simulink model "Supported_and_unsupported_combinations"  (Simulink 7.8)
settings: Solver=ode15s  StartTime=0.0  StopTime=inf  MaxStep=0.2  RelTol=1e-3
undefined symbols (not defined in the file): Engine, Engine1, Engine2, Engine3, Engine4, Engine5, Engine6, Engine7, Engine8, Engine9
libraries: sFunctionBlocks x32
(part 1 of 4)
settings Model: Creator=e675225  LastModifiedBy=e675225
settings DebuggingCC: UnconnectedLineMsg=none

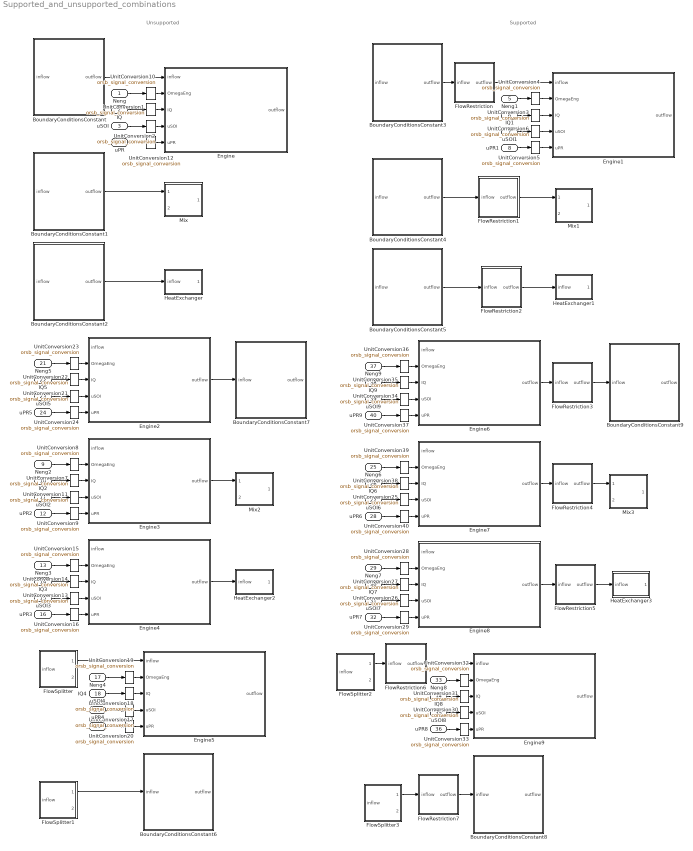
== system Supported_and_unsupported_combinations ==
  note: Unsupported
  note: Supported
  Neng : Inport
  IQ : Inport  Port=2
  uSOI : Inport  Tag=actuator  Port=3
  uPR : Inport  Port=4
  Neng1 : Inport  Port=5
  IQ1 : Inport  Port=6
  uSOI1 : Inport  Tag=actuator  Port=7
  uPR1 : Inport  Port=8
  Neng2 : Inport  Port=9
  IQ2 : Inport  Port=10
  uSOI2 : Inport  Tag=actuator  Port=11
  uPR2 : Inport  Port=12
  Neng3 : Inport  Port=13
  IQ3 : Inport  Port=14
  uSOI3 : Inport  Tag=actuator  Port=15
  uPR3 : Inport  Port=16
  Neng4 : Inport  Port=17
  IQ4 : Inport  Port=18
  uSOI4 : Inport  Tag=actuator  Port=19
  uPR4 : Inport  Port=20
  Neng5 : Inport  Port=21
  IQ5 : Inport  Port=22
  uSOI5 : Inport  Tag=actuator  Port=23
  uPR5 : Inport  Port=24
  Neng6 : Inport  Port=25
  IQ6 : Inport  Port=26
  uSOI6 : Inport  Tag=actuator  Port=27
  uPR6 : Inport  Port=28
  Neng7 : Inport  Port=29
  IQ7 : Inport  Port=30
  uSOI7 : Inport  Tag=actuator  Port=31
  uPR7 : Inport  Port=32
  Neng8 : Inport  Port=33
  IQ8 : Inport  Port=34
  uSOI8 : Inport  Tag=actuator  Port=35
  uPR8 : Inport  Port=36
  Neng9 : Inport  Port=37
  IQ9 : Inport  Port=38
  uSOI9 : Inport  Tag=actuator  Port=39
  uPR9 : Inport  Port=40
  BoundaryConditionsConstant : Subsystem  mask(amb_conditions){XO2bc=0.231362, Tbc=293, Pbc=1e5}
      mask prompts: XO2bc "<b>XO2bc:</b> boundary condition oxygen mass fraction [-]"; Tbc "<b>Tbc:</b> boundary condition temperature [K]"; Pbc "<b>Pbc:</b> boundary condition pressure [Pa]"
      mask Display:
      | plot([0], [-0.5])
      | plot([1], [0.5])
      | plot((0.1:0.01:0.87), sqrt(0.8*((0.1:0.01:0.87)-0.1)-((0.1:0.01:0.87)-0.1).^2))
      | plot((0.1:0.01:0.87), -sqrt(0.8*((0.1:0.01:0.87)-0.1)-((0.1:0.01:0.87)-0.1).^2))
      | plot([0.87 0.95], sqrt(0.8*((0.87)-0.1)-((0.87)-0.1).^2)*[1 1])
      | plot([0.87 0.95], -sqrt(0.8*((0.87)-0.1)-((0.87)-0.1).^2)*[1 1])
  BoundaryConditionsConstant1 : Subsystem  mask(amb_conditions){XO2bc=0.231362, Tbc=293, Pbc=1e5}
      mask prompts: XO2bc "<b>XO2bc:</b> boundary condition oxygen mass fraction [-]"; Tbc "<b>Tbc:</b> boundary condition temperature [K]"; Pbc "<b>Pbc:</b> boundary condition pressure [Pa]"
      mask Display:
      | plot([0], [-0.5])
      | plot([1], [0.5])
      | plot((0.1:0.01:0.87), sqrt(0.8*((0.1:0.01:0.87)-0.1)-((0.1:0.01:0.87)-0.1).^2))
      | plot((0.1:0.01:0.87), -sqrt(0.8*((0.1:0.01:0.87)-0.1)-((0.1:0.01:0.87)-0.1).^2))
      | plot([0.87 0.95], sqrt(0.8*((0.87)-0.1)-((0.87)-0.1).^2)*[1 1])
      | plot([0.87 0.95], -sqrt(0.8*((0.87)-0.1)-((0.87)-0.1).^2)*[1 1])
  BoundaryConditionsConstant2 : Subsystem  mask(amb_conditions){XO2bc=0.231362, Tbc=293, Pbc=1e5}
      mask prompts: XO2bc "<b>XO2bc:</b> boundary condition oxygen mass fraction [-]"; Tbc "<b>Tbc:</b> boundary condition temperature [K]"; Pbc "<b>Pbc:</b> boundary condition pressure [Pa]"
      mask Display:
      | plot([0], [-0.5])
      | plot([1], [0.5])
      | plot((0.1:0.01:0.87), sqrt(0.8*((0.1:0.01:0.87)-0.1)-((0.1:0.01:0.87)-0.1).^2))
      | plot((0.1:0.01:0.87), -sqrt(0.8*((0.1:0.01:0.87)-0.1)-((0.1:0.01:0.87)-0.1).^2))
      | plot([0.87 0.95], sqrt(0.8*((0.87)-0.1)-((0.87)-0.1).^2)*[1 1])
      | plot([0.87 0.95], -sqrt(0.8*((0.87)-0.1)-((0.87)-0.1).^2)*[1 1])
  BoundaryConditionsConstant3 : Subsystem  mask(amb_conditions){XO2bc=0.231362, Tbc=293, Pbc=1e5}
      mask prompts: XO2bc "<b>XO2bc:</b> boundary condition oxygen mass fraction [-]"; Tbc "<b>Tbc:</b> boundary condition temperature [K]"; Pbc "<b>Pbc:</b> boundary condition pressure [Pa]"
      mask Display:
      | plot([0], [-0.5])
      | plot([1], [0.5])
      | plot((0.1:0.01:0.87), sqrt(0.8*((0.1:0.01:0.87)-0.1)-((0.1:0.01:0.87)-0.1).^2))
      | plot((0.1:0.01:0.87), -sqrt(0.8*((0.1:0.01:0.87)-0.1)-((0.1:0.01:0.87)-0.1).^2))
      | plot([0.87 0.95], sqrt(0.8*((0.87)-0.1)-((0.87)-0.1).^2)*[1 1])
      | plot([0.87 0.95], -sqrt(0.8*((0.87)-0.1)-((0.87)-0.1).^2)*[1 1])
  BoundaryConditionsConstant4 : Subsystem  mask(amb_conditions){XO2bc=0.231362, Tbc=293, Pbc=1e5}
      mask prompts: XO2bc "<b>XO2bc:</b> boundary condition oxygen mass fraction [-]"; Tbc "<b>Tbc:</b> boundary condition temperature [K]"; Pbc "<b>Pbc:</b> boundary condition pressure [Pa]"
      mask Display:
      | plot([0], [-0.5])
      | plot([1], [0.5])
      | plot((0.1:0.01:0.87), sqrt(0.8*((0.1:0.01:0.87)-0.1)-((0.1:0.01:0.87)-0.1).^2))
      | plot((0.1:0.01:0.87), -sqrt(0.8*((0.1:0.01:0.87)-0.1)-((0.1:0.01:0.87)-0.1).^2))
      | plot([0.87 0.95], sqrt(0.8*((0.87)-0.1)-((0.87)-0.1).^2)*[1 1])
      | plot([0.87 0.95], -sqrt(0.8*((0.87)-0.1)-((0.87)-0.1).^2)*[1 1])
  BoundaryConditionsConstant5 : Subsystem  mask(amb_conditions){XO2bc=0.231362, Tbc=293, Pbc=1e5}
      mask prompts: XO2bc "<b>XO2bc:</b> boundary condition oxygen mass fraction [-]"; Tbc "<b>Tbc:</b> boundary condition temperature [K]"; Pbc "<b>Pbc:</b> boundary condition pressure [Pa]"
      mask Display:
      | plot([0], [-0.5])
      | plot([1], [0.5])
      | plot((0.1:0.01:0.87), sqrt(0.8*((0.1:0.01:0.87)-0.1)-((0.1:0.01:0.87)-0.1).^2))
      | plot((0.1:0.01:0.87), -sqrt(0.8*((0.1:0.01:0.87)-0.1)-((0.1:0.01:0.87)-0.1).^2))
      | plot([0.87 0.95], sqrt(0.8*((0.87)-0.1)-((0.87)-0.1).^2)*[1 1])
      | plot([0.87 0.95], -sqrt(0.8*((0.87)-0.1)-((0.87)-0.1).^2)*[1 1])
  BoundaryConditionsConstant6 : Subsystem  mask(amb_conditions){XO2bc=0.231362, Tbc=293, Pbc=1e5}
      mask prompts: XO2bc "<b>XO2bc:</b> boundary condition oxygen mass fraction [-]"; Tbc "<b>Tbc:</b> boundary condition temperature [K]"; Pbc "<b>Pbc:</b> boundary condition pressure [Pa]"
      mask Display:
      | plot([0], [-0.5])
      | plot([1], [0.5])
      | plot((0.1:0.01:0.87), sqrt(0.8*((0.1:0.01:0.87)-0.1)-((0.1:0.01:0.87)-0.1).^2))
      | plot((0.1:0.01:0.87), -sqrt(0.8*((0.1:0.01:0.87)-0.1)-((0.1:0.01:0.87)-0.1).^2))
      | plot([0.87 0.95], sqrt(0.8*((0.87)-0.1)-((0.87)-0.1).^2)*[1 1])
      | plot([0.87 0.95], -sqrt(0.8*((0.87)-0.1)-((0.87)-0.1).^2)*[1 1])
  BoundaryConditionsConstant7 : Subsystem  mask(amb_conditions){XO2bc=0.231362, Tbc=293, Pbc=1e5}
      mask prompts: XO2bc "<b>XO2bc:</b> boundary condition oxygen mass fraction [-]"; Tbc "<b>Tbc:</b> boundary condition temperature [K]"; Pbc "<b>Pbc:</b> boundary condition pressure [Pa]"
      mask Display:
      | plot([0], [-0.5])
      | plot([1], [0.5])
      | plot((0.1:0.01:0.87), sqrt(0.8*((0.1:0.01:0.87)-0.1)-((0.1:0.01:0.87)-0.1).^2))
      | plot((0.1:0.01:0.87), -sqrt(0.8*((0.1:0.01:0.87)-0.1)-((0.1:0.01:0.87)-0.1).^2))
      | plot([0.87 0.95], sqrt(0.8*((0.87)-0.1)-((0.87)-0.1).^2)*[1 1])
      | plot([0.87 0.95], -sqrt(0.8*((0.87)-0.1)-((0.87)-0.1).^2)*[1 1])
  BoundaryConditionsConstant8 : Subsystem  mask(amb_conditions){XO2bc=0.231362, Tbc=293, Pbc=1e5}
      mask prompts: XO2bc "<b>XO2bc:</b> boundary condition oxygen mass fraction [-]"; Tbc "<b>Tbc:</b> boundary condition temperature [K]"; Pbc "<b>Pbc:</b> boundary condition pressure [Pa]"
      mask Display:
      | plot([0], [-0.5])
      | plot([1], [0.5])
      | plot((0.1:0.01:0.87), sqrt(0.8*((0.1:0.01:0.87)-0.1)-((0.1:0.01:0.87)-0.1).^2))
      | plot((0.1:0.01:0.87), -sqrt(0.8*((0.1:0.01:0.87)-0.1)-((0.1:0.01:0.87)-0.1).^2))
      | plot([0.87 0.95], sqrt(0.8*((0.87)-0.1)-((0.87)-0.1).^2)*[1 1])
      | plot([0.87 0.95], -sqrt(0.8*((0.87)-0.1)-((0.87)-0.1).^2)*[1 1])
  BoundaryConditionsConstant9 : Subsystem  mask(amb_conditions){XO2bc=0.231362, Tbc=293, Pbc=1e5}
      mask prompts: XO2bc "<b>XO2bc:</b> boundary condition oxygen mass fraction [-]"; Tbc "<b>Tbc:</b> boundary condition temperature [K]"; Pbc "<b>Pbc:</b> boundary condition pressure [Pa]"
      mask Display:
      | plot([0], [-0.5])
      | plot([1], [0.5])
      | plot((0.1:0.01:0.87), sqrt(0.8*((0.1:0.01:0.87)-0.1)-((0.1:0.01:0.87)-0.1).^2))
      | plot((0.1:0.01:0.87), -sqrt(0.8*((0.1:0.01:0.87)-0.1)-((0.1:0.01:0.87)-0.1).^2))
      | plot([0.87 0.95], sqrt(0.8*((0.87)-0.1)-((0.87)-0.1).^2)*[1 1])
      | plot([0.87 0.95], -sqrt(0.8*((0.87)-0.1)-((0.87)-0.1).^2)*[1 1])
  Engine : Subsystem  mask(engine_subsys){setOutportFuel_Massflow=off, nameOutportFuel_Massflow=Fuel_Massflow_Engine, setOutportEngine_Speed=off, nameOutportEngine_Speed=Omega_Engine, setOutportCylinder_Pressure=off, nameOutportCylinder_Pressure=Pressure_in_cylinder_Engine, blockName=Engine}
      mask prompts: setOutportFuel_Massflow "readout fuel mass flow [kg/s]"; nameOutportFuel_Massflow "variable name to readout fuel mass flow"; setOutportEngine_Speed "readout engine speed [rad/s]"; nameOutportEngine_Speed "variable name to readout engine speed"; setOutportCylinder_Pressure "readout cylinder pressure [Pa]"; nameOutportCylinder_Pressure "variable name to readout cylinder pressure"; blockName "name of readout block (internal use only)"
      mask init:
      | %Speed icon
      | if setOutportEngine_Speed
      |     r = 0.08;
      |     xCenter = 0.5;
      |     yCenter = 0.2;
      |     xSpeed1 = [0.53 0.5 0.53];                          ySpeed1 = yCenter - 1*(r + [0.04 0 -0.04]);
      |     xSpeed2 = ((xCenter-r) : 0.001 :(xCenter + r)); ySpeed2 = yCenter + 1*sqrt(abs(r^2-(xSpeed2-xCenter).^2));
      |     xSpeed3 = xSpeed2;                              ySpeed3 = yCenter - 1*sqrt(abs(r^2-(xSpeed3-xCenter).^2));
      | else
      |     xSpeed1 = 0;   ySpeed1 = 0;
      |     xSpeed2 = 0;   ySpeed2 = 0;
      |     xSpeed3 = 0;   ySpeed3 = 0;
      | end
      | 
      | 
      | %Massflow icon
      | if setOutportFuel_Massflow
      |     xFlow1 = [0.45 0.45]; yFlow1 = [0.95 0.85];
      |     xFlow2 = [0.55 0.55];	yFlow2 = yFlow1;
      |     xFlow3 = [0.5 0.5];	yFlow3 = [0.97 0.83];
      |     xFlow4 = [0.49 0.5 0.51];    yFlow4 = [0.87 0.83 0.87];
      | else
      |     xFlow1 = 0;    yFlow1 = 0;
      |     xFlow2 = 0;    yFlow2 = 0;
      |     xFlow3 = 0;    yFlow3 = 0;
      |     xFlow4 = 0;    yFlow4 = 0;
      | end
      | 
      | 
      | %Pressure icon
      | if setOutportCylinder_Pressure
      |     r = 0.06;
      |     xCenter = 0.5;
      |     yCenter = 1.1;
      |     xPress1 = [xCenter-r xCenter+r];                yPress1 = [yCenter-r yCenter+r];
      |     xPress2 = [xCenter+r-r/4 xCenter+r xCenter+r];  yPress2 = [yCenter+r yCenter+r yCenter+r-r/4];
      |     xPress3 = ((xCenter-r) : 0.001 :(xCenter + r)); yPress3 = yCenter + sqrt(abs(r^2-(xPress3-xCenter).^2));
      |     xPress4 = xPress3;                              yPress4 = yCenter - sqrt(abs(r^2-(xPress4-xCenter).^2));
      | else
      |     xPress1 = 0;   yPress1 = 0;
      |     xPress2 = 0;   yPress2 = 0;
      |     xPress3 = 0;   yPress3 = 0;
      |     xPress4 = 0;   yPress4 = 0;
      | end
      settings: CopyFcn=|
      | set_param(gcb, 'blockName', get_param(gcb, 'Name'))
      | set_param(gcb, 'setOutportFuel_Massflow', 'off')
      | set_param(gcb, 'nameOutportFuel_Massflow', ['Fuel_Massflow_' get_param(gcb, 'blockName')])
      | set_param(gcb, 'setOutportEngine_Speed', 'off')
      | set_param(gcb, 'nameOutportEngine_Speed', ['Omega_' get_param(gcb, 'blockName')])
      | set_param(gcb, 'setOutportCylinder_Pressure', 'off')
      | set_param(gcb, 'nameOutportCylinder_Pressure', ['Pressure_in_cylinder_' get_param(gcb, 'blockName')])
      settings: NameChangeFcn=|
      | %if variable name is default change this name on name change of block
      | 
      | 
      | if strcmp(get_param(gcb, 'nameOutportFuel_Massflow'), [ 'Fuel_Massflow_' get_param(gcb, 'blockName') ])
      | set_param(gcb, 'nameOutportFuel_Massflow', ['Fuel_Massflow_' get_param(gcb, 'Name')])
      | end
      | 
      | 
      | 
      | 
      | if strcmp(get_param(gcb, 'nameOutportEngine_Speed'), [ 'Omega_' get_param(gcb, 'blockName') ])
      | set_param(gcb, 'nameOutportEngine_Speed', ['Omega_' get_param(gcb, 'Name')])
      | end
      | 
      | 
      | set_param(gcb, 'blockName', get_param(gcb, 'Name'))
      mask CallbackString:
      | en = get_param(gcb,'MaskEnables');
      | 
      | switch get_param(gcb,'setOutportFuel_Massflow')
      | 
      |     case 'on'
      |         en{2} = 'on';
      |     case 'off'
      |         en{2} = 'off';
      | end
      | 
      | set_param(gcb,'MaskEnables',en)|%% Check for empty strings
      | if isempty(strtrim(get_param(gcb, 'nameOutportFuel_Massflow')))
      |     set_param(gcb, 'nameOutportFuel_Massflow', ['Fuel_Massflow_' get_param(gcb, 'Name')])
      |     error('Empty string for readout variable not allowed')
      | end
      | 
      | 
      | %% Check for repeated outport names
      | checkOutportName('nameOutportFuel_Massflow', 'Fuel_Massflow')|en = get_param(gcb,'MaskEnables');
      | 
      | switch get_param(gcb,'setOutportEngine_Speed')
      | 
      |     case 'on'
      |         en{4} = 'on';
      |     case 'off'
      |         en{4} = 'off';
      | end
      | 
      | set_param(gcb,'MaskEnables',en)|%% Check for empty strings
      | if isempty(strtrim(get_param(gcb, 'nameOutportEngine_Speed')))
      |     set_param(gcb, 'nameOutportEngine_Speed', ['Engine_Speed_' get_param(gcb, 'Name')])
      |     error('Empty string for readout variable not allowed')
      | end
      | 
      | 
      | %% Check for repeated outport names
      | checkOutportName('nameOutportEngine_Speed', 'Engine_Speed')|en = get_param(gcb,'MaskEnables');
      | 
      | switch get_param(gcb,'setOutportCylinder_Pressure')
      | 
      |     case 'on'
      |         en{6} = 'on';
      |     case 'off'
      |         en{6} = 'off';
      | end
      | 
      | set_param(gcb,'MaskEnables',en)|%% Check for empty strings
      | if isempty(strtrim(get_param(gcb, 'nameOutportFuel_Massflow')))
      |     set_param(gcb, 'nameOutportFuel_Massflow', ['Fuel_Massflow_' get_param(gcb, 'Name')])
      |     error('Empty string for readout variable not allowed')
      | end
      | 
      | 
      | %% Check for repeated outport names
      | checkOutportName('nameOutportFuel_Massflow', 'Fuel_Massflow')|
      mask Display:
      | plot([-0.1], [-0.1])
      | plot([1.1], [1.1])
      | plot([0.18,0.18],[0,1])
      | plot([0.21,0.21],[0,1])
      | plot([0.82,0.82],[0,1])
      | plot([0.79,0.79],[0,1])
      | plot([0.22,0.22,0.3, 0.7, 0.78, 0.78, 0.22],[0.8, 0.4, 0.35, 0.35, 0.4,0.8,0.8])
      | plot([0.21,0.79],[0.7,0.7])
      | plot([0.21,0.79],[0.66,0.66])
      | plot([0.21,0.79],[0.7,0.7])
      | plot([0.47,0.6],[0.35,0])
      | plot([0.53,0.66],[0.35,0])
      | 
      | color('green');
      | plot(xSpeed1, ySpeed1)
      | plot(xSpeed2, ySpeed2)
      | plot(xSpeed3, ySpeed3)
      | 
      | color('magenta');
      | plot(xFlow1, yFlow1)
      | plot(xFlow2, yFlow2)
      | plot(xFlow3, yFlow3)
      | plot(xFlow4, yFlow4)
      | 
      | color('blue');
      | plot(xPress1, yPress1)
      | plot(xPress2, yPress2)
      | plot(xPress3, yPress3)
      | plot(xPress4, yPress4)
  Engine1 : Subsystem  mask(engine_subsys){setOutportFuel_Massflow=off, nameOutportFuel_Massflow=Fuel_Massflow_Engine1, setOutportEngine_Speed=off, nameOutportEngine_Speed=Omega_Engine1, setOutportCylinder_Pressure=off, nameOutportCylinder_Pressure=Pressure_in_cylinder_Engine1, blockName=Engine1}
      mask prompts: setOutportFuel_Massflow "readout fuel mass flow [kg/s]"; nameOutportFuel_Massflow "variable name to readout fuel mass flow"; setOutportEngine_Speed "readout engine speed [rad/s]"; nameOutportEngine_Speed "variable name to readout engine speed"; setOutportCylinder_Pressure "readout cylinder pressure [Pa]"; nameOutportCylinder_Pressure "variable name to readout cylinder pressure"; blockName "name of readout block (internal use only)"
      mask init: same as Supported_and_unsupported_combinations/Engine
      settings: CopyFcn=|
      | set_param(gcb, 'blockName', get_param(gcb, 'Name'))
      | set_param(gcb, 'setOutportFuel_Massflow', 'off')
      | set_param(gcb, 'nameOutportFuel_Massflow', ['Fuel_Massflow_' get_param(gcb, 'blockName')])
      | set_param(gcb, 'setOutportEngine_Speed', 'off')
      | set_param(gcb, 'nameOutportEngine_Speed', ['Omega_' get_param(gcb, 'blockName')])
      | set_param(gcb, 'setOutportCylinder_Pressure', 'off')
      | set_param(gcb, 'nameOutportCylinder_Pressure', ['Pressure_in_cylinder_' get_param(gcb, 'blockName')])
      settings: NameChangeFcn=|
      | %if variable name is default change this name on name change of block
      | 
      | 
      | if strcmp(get_param(gcb, 'nameOutportFuel_Massflow'), [ 'Fuel_Massflow_' get_param(gcb, 'blockName') ])
      | set_param(gcb, 'nameOutportFuel_Massflow', ['Fuel_Massflow_' get_param(gcb, 'Name')])
      | end
      | 
      | 
      | 
      | 
      | if strcmp(get_param(gcb, 'nameOutportEngine_Speed'), [ 'Omega_' get_param(gcb, 'blockName') ])
      | set_param(gcb, 'nameOutportEngine_Speed', ['Omega_' get_param(gcb, 'Name')])
      | end
      | 
      | 
      | set_param(gcb, 'blockName', get_param(gcb, 'Name'))
      mask CallbackString:
      | en = get_param(gcb,'MaskEnables');
      | 
      | switch get_param(gcb,'setOutportFuel_Massflow')
      | 
      |     case 'on'
      |         en{2} = 'on';
      |     case 'off'
      |         en{2} = 'off';
      | end
      | 
      | set_param(gcb,'MaskEnables',en)|%% Check for empty strings
      | if isempty(strtrim(get_param(gcb, 'nameOutportFuel_Massflow')))
      |     set_param(gcb, 'nameOutportFuel_Massflow', ['Fuel_Massflow_' get_param(gcb, 'Name')])
      |     error('Empty string for readout variable not allowed')
      | end
      | 
      | 
      | %% Check for repeated outport names
      | checkOutportName('nameOutportFuel_Massflow', 'Fuel_Massflow')|en = get_param(gcb,'MaskEnables');
      | 
      | switch get_param(gcb,'setOutportEngine_Speed')
      | 
      |     case 'on'
      |         en{4} = 'on';
      |     case 'off'
      |         en{4} = 'off';
      | end
      | 
      | set_param(gcb,'MaskEnables',en)|%% Check for empty strings
      | if isempty(strtrim(get_param(gcb, 'nameOutportEngine_Speed')))
      |     set_param(gcb, 'nameOutportEngine_Speed', ['Engine_Speed_' get_param(gcb, 'Name')])
      |     error('Empty string for readout variable not allowed')
      | end
      | 
      | 
      | %% Check for repeated outport names
      | checkOutportName('nameOutportEngine_Speed', 'Engine_Speed')|en = get_param(gcb,'MaskEnables');
      | 
      | switch get_param(gcb,'setOutportCylinder_Pressure')
      | 
      |     case 'on'
      |         en{6} = 'on';
      |     case 'off'
      |         en{6} = 'off';
      | end
      | 
      | set_param(gcb,'MaskEnables',en)|%% Check for empty strings
      | if isempty(strtrim(get_param(gcb, 'nameOutportFuel_Massflow')))
      |     set_param(gcb, 'nameOutportFuel_Massflow', ['Fuel_Massflow_' get_param(gcb, 'Name')])
      |     error('Empty string for readout variable not allowed')
      | end
      | 
      | 
      | %% Check for repeated outport names
      | checkOutportName('nameOutportFuel_Massflow', 'Fuel_Massflow')|
      mask Display:
      | plot([-0.1], [-0.1])
      | plot([1.1], [1.1])
      | plot([0.18,0.18],[0,1])
      | plot([0.21,0.21],[0,1])
      | plot([0.82,0.82],[0,1])
      | plot([0.79,0.79],[0,1])
      | plot([0.22,0.22,0.3, 0.7, 0.78, 0.78, 0.22],[0.8, 0.4, 0.35, 0.35, 0.4,0.8,0.8])
      | plot([0.21,0.79],[0.7,0.7])
      | plot([0.21,0.79],[0.66,0.66])
      | plot([0.21,0.79],[0.7,0.7])
      | plot([0.47,0.6],[0.35,0])
      | plot([0.53,0.66],[0.35,0])
      | 
      | color('green');
      | plot(xSpeed1, ySpeed1)
      | plot(xSpeed2, ySpeed2)
      | plot(xSpeed3, ySpeed3)
      | 
      | color('magenta');
      | plot(xFlow1, yFlow1)
      | plot(xFlow2, yFlow2)
      | plot(xFlow3, yFlow3)
      | plot(xFlow4, yFlow4)
      | 
      | color('blue');
      | plot(xPress1, yPress1)
      | plot(xPress2, yPress2)
      | plot(xPress3, yPress3)
      | plot(xPress4, yPress4)
  Engine2 : Subsystem  mask(engine_subsys){setOutportFuel_Massflow=off, nameOutportFuel_Massflow=Fuel_Massflow_Engine2, setOutportEngine_Speed=off, nameOutportEngine_Speed=Omega_Engine2, setOutportCylinder_Pressure=off, nameOutportCylinder_Pressure=Pressure_in_cylinder_Engine5, blockName=Engine2}
      mask prompts: setOutportFuel_Massflow "readout fuel mass flow [kg/s]"; nameOutportFuel_Massflow "variable name to readout fuel mass flow"; setOutportEngine_Speed "readout engine speed [rad/s]"; nameOutportEngine_Speed "variable name to readout engine speed"; setOutportCylinder_Pressure "readout cylinder pressure [Pa]"; nameOutportCylinder_Pressure "variable name to readout cylinder pressure"; blockName "name of readout block (internal use only)"
      mask init: same as Supported_and_unsupported_combinations/Engine
      settings: CopyFcn=|
      | set_param(gcb, 'blockName', get_param(gcb, 'Name'))
      | set_param(gcb, 'setOutportFuel_Massflow', 'off')
      | set_param(gcb, 'nameOutportFuel_Massflow', ['Fuel_Massflow_' get_param(gcb, 'blockName')])
      | set_param(gcb, 'setOutportEngine_Speed', 'off')
      | set_param(gcb, 'nameOutportEngine_Speed', ['Omega_' get_param(gcb, 'blockName')])
      | set_param(gcb, 'setOutportCylinder_Pressure', 'off')
      | set_param(gcb, 'nameOutportCylinder_Pressure', ['Pressure_in_cylinder_' get_param(gcb, 'blockName')])
      settings: NameChangeFcn=|
      | %if variable name is default change this name on name change of block
      | 
      | 
      | if strcmp(get_param(gcb, 'nameOutportFuel_Massflow'), [ 'Fuel_Massflow_' get_param(gcb, 'blockName') ])
      | set_param(gcb, 'nameOutportFuel_Massflow', ['Fuel_Massflow_' get_param(gcb, 'Name')])
      | end
      | 
      | 
      | 
      | 
      | if strcmp(get_param(gcb, 'nameOutportEngine_Speed'), [ 'Omega_' get_param(gcb, 'blockName') ])
      | set_param(gcb, 'nameOutportEngine_Speed', ['Omega_' get_param(gcb, 'Name')])
      | end
      | 
      | 
      | set_param(gcb, 'blockName', get_param(gcb, 'Name'))
      mask CallbackString:
      | en = get_param(gcb,'MaskEnables');
      | 
      | switch get_param(gcb,'setOutportFuel_Massflow')
      | 
      |     case 'on'
      |         en{2} = 'on';
      |     case 'off'
      |         en{2} = 'off';
      | end
      | 
      | set_param(gcb,'MaskEnables',en)|%% Check for empty strings
      | if isempty(strtrim(get_param(gcb, 'nameOutportFuel_Massflow')))
      |     set_param(gcb, 'nameOutportFuel_Massflow', ['Fuel_Massflow_' get_param(gcb, 'Name')])
      |     error('Empty string for readout variable not allowed')
      | end
      | 
      | 
      | %% Check for repeated outport names
      | checkOutportName('nameOutportFuel_Massflow', 'Fuel_Massflow')|en = get_param(gcb,'MaskEnables');
      | 
      | switch get_param(gcb,'setOutportEngine_Speed')
      | 
      |     case 'on'
      |         en{4} = 'on';
      |     case 'off'
      |         en{4} = 'off';
      | end
      | 
      | set_param(gcb,'MaskEnables',en)|%% Check for empty strings
      | if isempty(strtrim(get_param(gcb, 'nameOutportEngine_Speed')))
      |     set_param(gcb, 'nameOutportEngine_Speed', ['Engine_Speed_' get_param(gcb, 'Name')])
      |     error('Empty string for readout variable not allowed')
      | end
      | 
      | 
      | %% Check for repeated outport names
      | checkOutportName('nameOutportEngine_Speed', 'Engine_Speed')|en = get_param(gcb,'MaskEnables');
      | 
      | switch get_param(gcb,'setOutportCylinder_Pressure')
      | 
      |     case 'on'
      |         en{6} = 'on';
      |     case 'off'
      |         en{6} = 'off';
      | end
      | 
      | set_param(gcb,'MaskEnables',en)|%% Check for empty strings
      | if isempty(strtrim(get_param(gcb, 'nameOutportFuel_Massflow')))
      |     set_param(gcb, 'nameOutportFuel_Massflow', ['Fuel_Massflow_' get_param(gcb, 'Name')])
      |     error('Empty string for readout variable not allowed')
      | end
      | 
      | 
      | %% Check for repeated outport names
      | checkOutportName('nameOutportFuel_Massflow', 'Fuel_Massflow')|
      mask Display:
      | plot([-0.1], [-0.1])
      | plot([1.1], [1.1])
      | plot([0.18,0.18],[0,1])
      | plot([0.21,0.21],[0,1])
      | plot([0.82,0.82],[0,1])
      | plot([0.79,0.79],[0,1])
      | plot([0.22,0.22,0.3, 0.7, 0.78, 0.78, 0.22],[0.8, 0.4, 0.35, 0.35, 0.4,0.8,0.8])
      | plot([0.21,0.79],[0.7,0.7])
      | plot([0.21,0.79],[0.66,0.66])
      | plot([0.21,0.79],[0.7,0.7])
      | plot([0.47,0.6],[0.35,0])
      | plot([0.53,0.66],[0.35,0])
      | 
      | color('green');
      | plot(xSpeed1, ySpeed1)
      | plot(xSpeed2, ySpeed2)
      | plot(xSpeed3, ySpeed3)
      | 
      | color('magenta');
      | plot(xFlow1, yFlow1)
      | plot(xFlow2, yFlow2)
      | plot(xFlow3, yFlow3)
      | plot(xFlow4, yFlow4)
      | 
      | color('blue');
      | plot(xPress1, yPress1)
      | plot(xPress2, yPress2)
      | plot(xPress3, yPress3)
      | plot(xPress4, yPress4)
  Engine3 : Subsystem  mask(engine_subsys){setOutportFuel_Massflow=off, nameOutportFuel_Massflow=Fuel_Massflow_Engine3, setOutportEngine_Speed=off, nameOutportEngine_Speed=Omega_Engine3, setOutportCylinder_Pressure=off, nameOutportCylinder_Pressure=Pressure_in_cylinder_Engine2, blockName=Engine3}
      mask prompts: setOutportFuel_Massflow "readout fuel mass flow [kg/s]"; nameOutportFuel_Massflow "variable name to readout fuel mass flow"; setOutportEngine_Speed "readout engine speed [rad/s]"; nameOutportEngine_Speed "variable name to readout engine speed"; setOutportCylinder_Pressure "readout cylinder pressure [Pa]"; nameOutportCylinder_Pressure "variable name to readout cylinder pressure"; blockName "name of readout block (internal use only)"
      mask init: same as Supported_and_unsupported_combinations/Engine
      settings: CopyFcn=|
      | set_param(gcb, 'blockName', get_param(gcb, 'Name'))
      | set_param(gcb, 'setOutportFuel_Massflow', 'off')
      | set_param(gcb, 'nameOutportFuel_Massflow', ['Fuel_Massflow_' get_param(gcb, 'blockName')])
      | set_param(gcb, 'setOutportEngine_Speed', 'off')
      | set_param(gcb, 'nameOutportEngine_Speed', ['Omega_' get_param(gcb, 'blockName')])
      | set_param(gcb, 'setOutportCylinder_Pressure', 'off')
      | set_param(gcb, 'nameOutportCylinder_Pressure', ['Pressure_in_cylinder_' get_param(gcb, 'blockName')])
      settings: NameChangeFcn=|
      | %if variable name is default change this name on name change of block
      | 
      | 
      | if strcmp(get_param(gcb, 'nameOutportFuel_Massflow'), [ 'Fuel_Massflow_' get_param(gcb, 'blockName') ])
      | set_param(gcb, 'nameOutportFuel_Massflow', ['Fuel_Massflow_' get_param(gcb, 'Name')])
      | end
      | 
      | 
      | 
      | 
      | if strcmp(get_param(gcb, 'nameOutportEngine_Speed'), [ 'Omega_' get_param(gcb, 'blockName') ])
      | set_param(gcb, 'nameOutportEngine_Speed', ['Omega_' get_param(gcb, 'Name')])
      | end
      | 
      | 
      | set_param(gcb, 'blockName', get_param(gcb, 'Name'))
      mask CallbackString:
      | en = get_param(gcb,'MaskEnables');
      | 
      | switch get_param(gcb,'setOutportFuel_Massflow')
      | 
      |     case 'on'
      |         en{2} = 'on';
      |     case 'off'
      |         en{2} = 'off';
      | end
      | 
      | set_param(gcb,'MaskEnables',en)|%% Check for empty strings
      | if isempty(strtrim(get_param(gcb, 'nameOutportFuel_Massflow')))
      |     set_param(gcb, 'nameOutportFuel_Massflow', ['Fuel_Massflow_' get_param(gcb, 'Name')])
      |     error('Empty string for readout variable not allowed')
      | end
      | 
      | 
      | %% Check for repeated outport names
      | checkOutportName('nameOutportFuel_Massflow', 'Fuel_Massflow')|en = get_param(gcb,'MaskEnables');
      | 
      | switch get_param(gcb,'setOutportEngine_Speed')
      | 
      |     case 'on'
      |         en{4} = 'on';
      |     case 'off'
      |         en{4} = 'off';
      | end
      | 
      | set_param(gcb,'MaskEnables',en)|%% Check for empty strings
      | if isempty(strtrim(get_param(gcb, 'nameOutportEngine_Speed')))
      |     set_param(gcb, 'nameOutportEngine_Speed', ['Engine_Speed_' get_param(gcb, 'Name')])
      |     error('Empty string for readout variable not allowed')
      | end
      | 
      | 
      | %% Check for repeated outport names
      | checkOutportName('nameOutportEngine_Speed', 'Engine_Speed')|en = get_param(gcb,'MaskEnables');
      | 
      | switch get_param(gcb,'setOutportCylinder_Pressure')
      | 
      |     case 'on'
      |         en{6} = 'on';
      |     case 'off'
      |         en{6} = 'off';
      | end
      | 
      | set_param(gcb,'MaskEnables',en)|%% Check for empty strings
      | if isempty(strtrim(get_param(gcb, 'nameOutportFuel_Massflow')))
      |     set_param(gcb, 'nameOutportFuel_Massflow', ['Fuel_Massflow_' get_param(gcb, 'Name')])
      |     error('Empty string for readout variable not allowed')
      | end
      | 
      | 
      | %% Check for repeated outport names
      | checkOutportName('nameOutportFuel_Massflow', 'Fuel_Massflow')|
      mask Display:
      | plot([-0.1], [-0.1])
      | plot([1.1], [1.1])
      | plot([0.18,0.18],[0,1])
      | plot([0.21,0.21],[0,1])
      | plot([0.82,0.82],[0,1])
      | plot([0.79,0.79],[0,1])
      | plot([0.22,0.22,0.3, 0.7, 0.78, 0.78, 0.22],[0.8, 0.4, 0.35, 0.35, 0.4,0.8,0.8])
      | plot([0.21,0.79],[0.7,0.7])
      | plot([0.21,0.79],[0.66,0.66])
      | plot([0.21,0.79],[0.7,0.7])
      | plot([0.47,0.6],[0.35,0])
      | plot([0.53,0.66],[0.35,0])
      | 
      | color('green');
      | plot(xSpeed1, ySpeed1)
      | plot(xSpeed2, ySpeed2)
      | plot(xSpeed3, ySpeed3)
      | 
      | color('magenta');
      | plot(xFlow1, yFlow1)
      | plot(xFlow2, yFlow2)
      | plot(xFlow3, yFlow3)
      | plot(xFlow4, yFlow4)
      | 
      | color('blue');
      | plot(xPress1, yPress1)
      | plot(xPress2, yPress2)
      | plot(xPress3, yPress3)
      | plot(xPress4, yPress4)
  Engine4 : Subsystem  mask(engine_subsys){setOutportFuel_Massflow=off, nameOutportFuel_Massflow=Fuel_Massflow_Engine4, setOutportEngine_Speed=off, nameOutportEngine_Speed=Omega_Engine4, setOutportCylinder_Pressure=off, nameOutportCylinder_Pressure=Pressure_in_cylinder_Engine3, blockName=Engine4}
      mask prompts: setOutportFuel_Massflow "readout fuel mass flow [kg/s]"; nameOutportFuel_Massflow "variable name to readout fuel mass flow"; setOutportEngine_Speed "readout engine speed [rad/s]"; nameOutportEngine_Speed "variable name to readout engine speed"; setOutportCylinder_Pressure "readout cylinder pressure [Pa]"; nameOutportCylinder_Pressure "variable name to readout cylinder pressure"; blockName "name of readout block (internal use only)"
      mask init: same as Supported_and_unsupported_combinations/Engine
      settings: CopyFcn=|
      | set_param(gcb, 'blockName', get_param(gcb, 'Name'))
      | set_param(gcb, 'setOutportFuel_Massflow', 'off')
      | set_param(gcb, 'nameOutportFuel_Massflow', ['Fuel_Massflow_' get_param(gcb, 'blockName')])
      | set_param(gcb, 'setOutportEngine_Speed', 'off')
      | set_param(gcb, 'nameOutportEngine_Speed', ['Omega_' get_param(gcb, 'blockName')])
      | set_param(gcb, 'setOutportCylinder_Pressure', 'off')
      | set_param(gcb, 'nameOutportCylinder_Pressure', ['Pressure_in_cylinder_' get_param(gcb, 'blockName')])
      settings: NameChangeFcn=|
      | %if variable name is default change this name on name change of block
      | 
      | 
      | if strcmp(get_param(gcb, 'nameOutportFuel_Massflow'), [ 'Fuel_Massflow_' get_param(gcb, 'blockName') ])
      | set_param(gcb, 'nameOutportFuel_Massflow', ['Fuel_Massflow_' get_param(gcb, 'Name')])
      | end
      | 
      | 
      | 
      | 
      | if strcmp(get_param(gcb, 'nameOutportEngine_Speed'), [ 'Omega_' get_param(gcb, 'blockName') ])
      | set_param(gcb, 'nameOutportEngine_Speed', ['Omega_' get_param(gcb, 'Name')])
      | end
      | 
      | 
      | set_param(gcb, 'blockName', get_param(gcb, 'Name'))
      mask CallbackString:
      | en = get_param(gcb,'MaskEnables');
      | 
      | switch get_param(gcb,'setOutportFuel_Massflow')
      | 
      |     case 'on'
      |         en{2} = 'on';
      |     case 'off'
      |         en{2} = 'off';
      | end
      | 
      | set_param(gcb,'MaskEnables',en)|%% Check for empty strings
      | if isempty(strtrim(get_param(gcb, 'nameOutportFuel_Massflow')))
      |     set_param(gcb, 'nameOutportFuel_Massflow', ['Fuel_Massflow_' get_param(gcb, 'Name')])
      |     error('Empty string for readout variable not allowed')
      | end
      | 
      | 
      | %% Check for repeated outport names
      | checkOutportName('nameOutportFuel_Massflow', 'Fuel_Massflow')|en = get_param(gcb,'MaskEnables');
      | 
      | switch get_param(gcb,'setOutportEngine_Speed')
      | 
      |     case 'on'
      |         en{4} = 'on';
      |     case 'off'
      |         en{4} = 'off';
      | end
      | 
      | set_param(gcb,'MaskEnables',en)|%% Check for empty strings
      | if isempty(strtrim(get_param(gcb, 'nameOutportEngine_Speed')))
      |     set_param(gcb, 'nameOutportEngine_Speed', ['Engine_Speed_' get_param(gcb, 'Name')])
      |     error('Empty string for readout variable not allowed')
      | end
      | 
      | 
      | %% Check for repeated outport names
      | checkOutportName('nameOutportEngine_Speed', 'Engine_Speed')|en = get_param(gcb,'MaskEnables');
      | 
      | switch get_param(gcb,'setOutportCylinder_Pressure')
      | 
      |     case 'on'
      |         en{6} = 'on';
      |     case 'off'
      |         en{6} = 'off';
      | end
      | 
      | set_param(gcb,'MaskEnables',en)|%% Check for empty strings
      | if isempty(strtrim(get_param(gcb, 'nameOutportFuel_Massflow')))
      |     set_param(gcb, 'nameOutportFuel_Massflow', ['Fuel_Massflow_' get_param(gcb, 'Name')])
      |     error('Empty string for readout variable not allowed')
      | end
      | 
      | 
      | %% Check for repeated outport names
      | checkOutportName('nameOutportFuel_Massflow', 'Fuel_Massflow')|
      mask Display:
      | plot([-0.1], [-0.1])
      | plot([1.1], [1.1])
      | plot([0.18,0.18],[0,1])
      | plot([0.21,0.21],[0,1])
      | plot([0.82,0.82],[0,1])
      | plot([0.79,0.79],[0,1])
      | plot([0.22,0.22,0.3, 0.7, 0.78, 0.78, 0.22],[0.8, 0.4, 0.35, 0.35, 0.4,0.8,0.8])
      | plot([0.21,0.79],[0.7,0.7])
      | plot([0.21,0.79],[0.66,0.66])
      | plot([0.21,0.79],[0.7,0.7])
      | plot([0.47,0.6],[0.35,0])
      | plot([0.53,0.66],[0.35,0])
      | 
      | color('green');
      | plot(xSpeed1, ySpeed1)
      | plot(xSpeed2, ySpeed2)
      | plot(xSpeed3, ySpeed3)
      | 
      | color('magenta');
      | plot(xFlow1, yFlow1)
      | plot(xFlow2, yFlow2)
      | plot(xFlow3, yFlow3)
      | plot(xFlow4, yFlow4)
      | 
      | color('blue');
      | plot(xPress1, yPress1)
      | plot(xPress2, yPress2)
      | plot(xPress3, yPress3)
      | plot(xPress4, yPress4)
  Engine5 : Subsystem  mask(engine_subsys){setOutportFuel_Massflow=off, nameOutportFuel_Massflow=Fuel_Massflow_Engine5, setOutportEngine_Speed=off, nameOutportEngine_Speed=Omega_Engine5, setOutportCylinder_Pressure=off, nameOutportCylinder_Pressure=Pressure_in_cylinder_Engine4, blockName=Engine5}
      mask prompts: setOutportFuel_Massflow "readout fuel mass flow [kg/s]"; nameOutportFuel_Massflow "variable name to readout fuel mass flow"; setOutportEngine_Speed "readout engine speed [rad/s]"; nameOutportEngine_Speed "variable name to readout engine speed"; setOutportCylinder_Pressure "readout cylinder pressure [Pa]"; nameOutportCylinder_Pressure "variable name to readout cylinder pressure"; blockName "name of readout block (internal use only)"
      mask init: same as Supported_and_unsupported_combinations/Engine
      settings: CopyFcn=|
      | set_param(gcb, 'blockName', get_param(gcb, 'Name'))
      | set_param(gcb, 'setOutportFuel_Massflow', 'off')
      | set_param(gcb, 'nameOutportFuel_Massflow', ['Fuel_Massflow_' get_param(gcb, 'blockName')])
      | set_param(gcb, 'setOutportEngine_Speed', 'off')
      | set_param(gcb, 'nameOutportEngine_Speed', ['Omega_' get_param(gcb, 'blockName')])
      | set_param(gcb, 'setOutportCylinder_Pressure', 'off')
      | set_param(gcb, 'nameOutportCylinder_Pressure', ['Pressure_in_cylinder_' get_param(gcb, 'blockName')])
      settings: NameChangeFcn=|
      | %if variable name is default change this name on name change of block
      | 
      | 
      | if strcmp(get_param(gcb, 'nameOutportFuel_Massflow'), [ 'Fuel_Massflow_' get_param(gcb, 'blockName') ])
      | set_param(gcb, 'nameOutportFuel_Massflow', ['Fuel_Massflow_' get_param(gcb, 'Name')])
      | end
      | 
      | 
      | 
      | 
      | if strcmp(get_param(gcb, 'nameOutportEngine_Speed'), [ 'Omega_' get_param(gcb, 'blockName') ])
      | set_param(gcb, 'nameOutportEngine_Speed', ['Omega_' get_param(gcb, 'Name')])
      | end
      | 
      | 
      | set_param(gcb, 'blockName', get_param(gcb, 'Name'))
      mask CallbackString:
      | en = get_param(gcb,'MaskEnables');
      | 
      | switch get_param(gcb,'setOutportFuel_Massflow')
      | 
      |     case 'on'
      |         en{2} = 'on';
      |     case 'off'
      |         en{2} = 'off';
      | end
      | 
      | set_param(gcb,'MaskEnables',en)|%% Check for empty strings
      | if isempty(strtrim(get_param(gcb, 'nameOutportFuel_Massflow')))
      |     set_param(gcb, 'nameOutportFuel_Massflow', ['Fuel_Massflow_' get_param(gcb, 'Name')])
      |     error('Empty string for readout variable not allowed')
      | end
      | 
      | 
      | %% Check for repeated outport names
      | checkOutportName('nameOutportFuel_Massflow', 'Fuel_Massflow')|en = get_param(gcb,'MaskEnables');
      | 
      | switch get_param(gcb,'setOutportEngine_Speed')
      | 
      |     case 'on'
      |         en{4} = 'on';
      |     case 'off'
      |         en{4} = 'off';
      | end
      | 
      | set_param(gcb,'MaskEnables',en)|%% Check for empty strings
      | if isempty(strtrim(get_param(gcb, 'nameOutportEngine_Speed')))
      |     set_param(gcb, 'nameOutportEngine_Speed', ['Engine_Speed_' get_param(gcb, 'Name')])
      |     error('Empty string for readout variable not allowed')
      | end
      | 
      | 
      | %% Check for repeated outport names
      | checkOutportName('nameOutportEngine_Speed', 'Engine_Speed')|en = get_param(gcb,'MaskEnables');
      | 
      | switch get_param(gcb,'setOutportCylinder_Pressure')
      | 
      |     case 'on'
      |         en{6} = 'on';
      |     case 'off'
      |         en{6} = 'off';
      | end
      | 
      | set_param(gcb,'MaskEnables',en)|%% Check for empty strings
      | if isempty(strtrim(get_param(gcb, 'nameOutportFuel_Massflow')))
      |     set_param(gcb, 'nameOutportFuel_Massflow', ['Fuel_Massflow_' get_param(gcb, 'Name')])
      |     error('Empty string for readout variable not allowed')
      | end
      | 
      | 
      | %% Check for repeated outport names
      | checkOutportName('nameOutportFuel_Massflow', 'Fuel_Massflow')|
      mask Display:
      | plot([-0.1], [-0.1])
      | plot([1.1], [1.1])
      | plot([0.18,0.18],[0,1])
      | plot([0.21,0.21],[0,1])
      | plot([0.82,0.82],[0,1])
      | plot([0.79,0.79],[0,1])
      | plot([0.22,0.22,0.3, 0.7, 0.78, 0.78, 0.22],[0.8, 0.4, 0.35, 0.35, 0.4,0.8,0.8])
      | plot([0.21,0.79],[0.7,0.7])
      | plot([0.21,0.79],[0.66,0.66])
      | plot([0.21,0.79],[0.7,0.7])
      | plot([0.47,0.6],[0.35,0])
      | plot([0.53,0.66],[0.35,0])
      | 
      | color('green');
      | plot(xSpeed1, ySpeed1)
      | plot(xSpeed2, ySpeed2)
      | plot(xSpeed3, ySpeed3)
      | 
      | color('magenta');
      | plot(xFlow1, yFlow1)
      | plot(xFlow2, yFlow2)
      | plot(xFlow3, yFlow3)
      | plot(xFlow4, yFlow4)
      | 
      | color('blue');
      | plot(xPress1, yPress1)
      | plot(xPress2, yPress2)
      | plot(xPress3, yPress3)
      | plot(xPress4, yPress4)
  Engine6 : Subsystem  mask(engine_subsys){setOutportFuel_Massflow=off, nameOutportFuel_Massflow=Fuel_Massflow_Engine6, setOutportEngine_Speed=off, nameOutportEngine_Speed=Omega_Engine6, setOutportCylinder_Pressure=off, nameOutportCylinder_Pressure=Pressure_in_cylinder_Engine6, blockName=Engine6}
      mask prompts: setOutportFuel_Massflow "readout fuel mass flow [kg/s]"; nameOutportFuel_Massflow "variable name to readout fuel mass flow"; setOutportEngine_Speed "readout engine speed [rad/s]"; nameOutportEngine_Speed "variable name to readout engine speed"; setOutportCylinder_Pressure "readout cylinder pressure [Pa]"; nameOutportCylinder_Pressure "variable name to readout cylinder pressure"; blockName "name of readout block (internal use only)"
      mask init: same as Supported_and_unsupported_combinations/Engine
      settings: CopyFcn=|
      | set_param(gcb, 'blockName', get_param(gcb, 'Name'))
      | set_param(gcb, 'setOutportFuel_Massflow', 'off')
      | set_param(gcb, 'nameOutportFuel_Massflow', ['Fuel_Massflow_' get_param(gcb, 'blockName')])
      | set_param(gcb, 'setOutportEngine_Speed', 'off')
      | set_param(gcb, 'nameOutportEngine_Speed', ['Omega_' get_param(gcb, 'blockName')])
      | set_param(gcb, 'setOutportCylinder_Pressure', 'off')
      | set_param(gcb, 'nameOutportCylinder_Pressure', ['Pressure_in_cylinder_' get_param(gcb, 'blockName')])
      settings: NameChangeFcn=|
      | %if variable name is default change this name on name change of block
      | 
      | 
      | if strcmp(get_param(gcb, 'nameOutportFuel_Massflow'), [ 'Fuel_Massflow_' get_param(gcb, 'blockName') ])
      | set_param(gcb, 'nameOutportFuel_Massflow', ['Fuel_Massflow_' get_param(gcb, 'Name')])
      | end
      | 
      | 
      | 
      | 
      | if strcmp(get_param(gcb, 'nameOutportEngine_Speed'), [ 'Omega_' get_param(gcb, 'blockName') ])
      | set_param(gcb, 'nameOutportEngine_Speed', ['Omega_' get_param(gcb, 'Name')])
      | end
      | 
      | 
      | set_param(gcb, 'blockName', get_param(gcb, 'Name'))
      mask CallbackString:
      | en = get_param(gcb,'MaskEnables');
      | 
      | switch get_param(gcb,'setOutportFuel_Massflow')
      | 
      |     case 'on'
      |         en{2} = 'on';
      |     case 'off'
      |         en{2} = 'off';
      | end
      | 
      | set_param(gcb,'MaskEnables',en)|%% Check for empty strings
      | if isempty(strtrim(get_param(gcb, 'nameOutportFuel_Massflow')))
      |     set_param(gcb, 'nameOutportFuel_Massflow', ['Fuel_Massflow_' get_param(gcb, 'Name')])
      |     error('Empty string for readout variable not allowed')
      | end
      | 
      | 
      | %% Check for repeated outport names
      | checkOutportName('nameOutportFuel_Massflow', 'Fuel_Massflow')|en = get_param(gcb,'MaskEnables');
      | 
      | switch get_param(gcb,'setOutportEngine_Speed')
      | 
      |     case 'on'
      |         en{4} = 'on';
      |     case 'off'
      |         en{4} = 'off';
      | end
      | 
      | set_param(gcb,'MaskEnables',en)|%% Check for empty strings
      | if isempty(strtrim(get_param(gcb, 'nameOutportEngine_Speed')))
      |     set_param(gcb, 'nameOutportEngine_Speed', ['Engine_Speed_' get_param(gcb, 'Name')])
      |     error('Empty string for readout variable not allowed')
      | end
      | 
      | 
      | %% Check for repeated outport names
      | checkOutportName('nameOutportEngine_Speed', 'Engine_Speed')|en = get_param(gcb,'MaskEnables');
      | 
      | switch get_param(gcb,'setOutportCylinder_Pressure')
      | 
      |     case 'on'
      |         en{6} = 'on';
      |     case 'off'
      |         en{6} = 'off';
      | end
      | 
      | set_param(gcb,'MaskEnables',en)|%% Check for empty strings
      | if isempty(strtrim(get_param(gcb, 'nameOutportFuel_Massflow')))
      |     set_param(gcb, 'nameOutportFuel_Massflow', ['Fuel_Massflow_' get_param(gcb, 'Name')])
      |     error('Empty string for readout variable not allowed')
      | end
      | 
      | 
      | %% Check for repeated outport names
      | checkOutportName('nameOutportFuel_Massflow', 'Fuel_Massflow')|
      mask Display:
      | plot([-0.1], [-0.1])
      | plot([1.1], [1.1])
      | plot([0.18,0.18],[0,1])
      | plot([0.21,0.21],[0,1])
      | plot([0.82,0.82],[0,1])
      | plot([0.79,0.79],[0,1])
      | plot([0.22,0.22,0.3, 0.7, 0.78, 0.78, 0.22],[0.8, 0.4, 0.35, 0.35, 0.4,0.8,0.8])
      | plot([0.21,0.79],[0.7,0.7])
      | plot([0.21,0.79],[0.66,0.66])
      | plot([0.21,0.79],[0.7,0.7])
      | plot([0.47,0.6],[0.35,0])
      | plot([0.53,0.66],[0.35,0])
      | 
      | color('green');
      | plot(xSpeed1, ySpeed1)
      | plot(xSpeed2, ySpeed2)
      | plot(xSpeed3, ySpeed3)
      | 
      | color('magenta');
      | plot(xFlow1, yFlow1)
      | plot(xFlow2, yFlow2)
      | plot(xFlow3, yFlow3)
      | plot(xFlow4, yFlow4)
      | 
      | color('blue');
      | plot(xPress1, yPress1)
      | plot(xPress2, yPress2)
      | plot(xPress3, yPress3)
      | plot(xPress4, yPress4)
  Engine7 : Subsystem  mask(engine_subsys){setOutportFuel_Massflow=off, nameOutportFuel_Massflow=Fuel_Massflow_Engine7, setOutportEngine_Speed=off, nameOutportEngine_Speed=Omega_Engine7, setOutportCylinder_Pressure=off, nameOutportCylinder_Pressure=Pressure_in_cylinder_Engine7, blockName=Engine7}
      mask prompts: setOutportFuel_Massflow "readout fuel mass flow [kg/s]"; nameOutportFuel_Massflow "variable name to readout fuel mass flow"; setOutportEngine_Speed "readout engine speed [rad/s]"; nameOutportEngine_Speed "variable name to readout engine speed"; setOutportCylinder_Pressure "readout cylinder pressure [Pa]"; nameOutportCylinder_Pressure "variable name to readout cylinder pressure"; blockName "name of readout block (internal use only)"
      mask init: same as Supported_and_unsupported_combinations/Engine
      settings: CopyFcn=|
      | set_param(gcb, 'blockName', get_param(gcb, 'Name'))
      | set_param(gcb, 'setOutportFuel_Massflow', 'off')
      | set_param(gcb, 'nameOutportFuel_Massflow', ['Fuel_Massflow_' get_param(gcb, 'blockName')])
      | set_param(gcb, 'setOutportEngine_Speed', 'off')
      | set_param(gcb, 'nameOutportEngine_Speed', ['Omega_' get_param(gcb, 'blockName')])
      | set_param(gcb, 'setOutportCylinder_Pressure', 'off')
      | set_param(gcb, 'nameOutportCylinder_Pressure', ['Pressure_in_cylinder_' get_param(gcb, 'blockName')])
      settings: NameChangeFcn=|
      | %if variable name is default change this name on name change of block
      | 
      | 
      | if strcmp(get_param(gcb, 'nameOutportFuel_Massflow'), [ 'Fuel_Massflow_' get_param(gcb, 'blockName') ])
      | set_param(gcb, 'nameOutportFuel_Massflow', ['Fuel_Massflow_' get_param(gcb, 'Name')])
      | end
      | 
      | 
      | 
      | 
      | if strcmp(get_param(gcb, 'nameOutportEngine_Speed'), [ 'Omega_' get_param(gcb, 'blockName') ])
      | set_param(gcb, 'nameOutportEngine_Speed', ['Omega_' get_param(gcb, 'Name')])
      | end
      | 
      | 
      | set_param(gcb, 'blockName', get_param(gcb, 'Name'))
      mask CallbackString:
      | en = get_param(gcb,'MaskEnables');
      | 
      | switch get_param(gcb,'setOutportFuel_Massflow')
      | 
      |     case 'on'
      |         en{2} = 'on';
      |     case 'off'
      |         en{2} = 'off';
      | end
      | 
      | set_param(gcb,'MaskEnables',en)|%% Check for empty strings
      | if isempty(strtrim(get_param(gcb, 'nameOutportFuel_Massflow')))
      |     set_param(gcb, 'nameOutportFuel_Massflow', ['Fuel_Massflow_' get_param(gcb, 'Name')])
      |     error('Empty string for readout variable not allowed')
      | end
      | 
      | 
      | %% Check for repeated outport names
      | checkOutportName('nameOutportFuel_Massflow', 'Fuel_Massflow')|en = get_param(gcb,'MaskEnables');
      | 
      | switch get_param(gcb,'setOutportEngine_Speed')
      | 
      |     case 'on'
      |         en{4} = 'on';
      |     case 'off'
      |         en{4} = 'off';
      | end
      | 
      | set_param(gcb,'MaskEnables',en)|%% Check for empty strings
      | if isempty(strtrim(get_param(gcb, 'nameOutportEngine_Speed')))
      |     set_param(gcb, 'nameOutportEngine_Speed', ['Engine_Speed_' get_param(gcb, 'Name')])
      |     error('Empty string for readout variable not allowed')
      | end
      | 
      | 
      | %% Check for repeated outport names
      | checkOutportName('nameOutportEngine_Speed', 'Engine_Speed')|en = get_param(gcb,'MaskEnables');
      | 
      | switch get_param(gcb,'setOutportCylinder_Pressure')
      | 
      |     case 'on'
      |         en{6} = 'on';
      |     case 'off'
      |         en{6} = 'off';
      | end
      | 
      | set_param(gcb,'MaskEnables',en)|%% Check for empty strings
      | if isempty(strtrim(get_param(gcb, 'nameOutportFuel_Massflow')))
      |     set_param(gcb, 'nameOutportFuel_Massflow', ['Fuel_Massflow_' get_param(gcb, 'Name')])
      |     error('Empty string for readout variable not allowed')
      | end
      | 
      | 
      | %% Check for repeated outport names
      | checkOutportName('nameOutportFuel_Massflow', 'Fuel_Massflow')|
      mask Display:
      | plot([-0.1], [-0.1])
      | plot([1.1], [1.1])
      | plot([0.18,0.18],[0,1])
      | plot([0.21,0.21],[0,1])
      | plot([0.82,0.82],[0,1])
      | plot([0.79,0.79],[0,1])
      | plot([0.22,0.22,0.3, 0.7, 0.78, 0.78, 0.22],[0.8, 0.4, 0.35, 0.35, 0.4,0.8,0.8])
      | plot([0.21,0.79],[0.7,0.7])
      | plot([0.21,0.79],[0.66,0.66])
      | plot([0.21,0.79],[0.7,0.7])
      | plot([0.47,0.6],[0.35,0])
      | plot([0.53,0.66],[0.35,0])
      | 
      | color('green');
      | plot(xSpeed1, ySpeed1)
      | plot(xSpeed2, ySpeed2)
      | plot(xSpeed3, ySpeed3)
      | 
      | color('magenta');
      | plot(xFlow1, yFlow1)
      | plot(xFlow2, yFlow2)
      | plot(xFlow3, yFlow3)
      | plot(xFlow4, yFlow4)
      | 
      | color('blue');
      | plot(xPress1, yPress1)
      | plot(xPress2, yPress2)
      | plot(xPress3, yPress3)
      | plot(xPress4, yPress4)
  Engine8 : Subsystem  mask(engine_subsys){setOutportFuel_Massflow=off, nameOutportFuel_Massflow=Fuel_Massflow_Engine8, setOutportEngine_Speed=off, nameOutportEngine_Speed=Omega_Engine8, setOutportCylinder_Pressure=off, nameOutportCylinder_Pressure=Pressure_in_cylinder_Engine8, blockName=Engine8}
      mask prompts: setOutportFuel_Massflow "readout fuel mass flow [kg/s]"; nameOutportFuel_Massflow "variable name to readout fuel mass flow"; setOutportEngine_Speed "readout engine speed [rad/s]"; nameOutportEngine_Speed "variable name to readout engine speed"; setOutportCylinder_Pressure "readout cylinder pressure [Pa]"; nameOutportCylinder_Pressure "variable name to readout cylinder pressure"; blockName "name of readout block (internal use only)"
      mask init: same as Supported_and_unsupported_combinations/Engine
      settings: CopyFcn=|
      | set_param(gcb, 'blockName', get_param(gcb, 'Name'))
      | set_param(gcb, 'setOutportFuel_Massflow', 'off')
      | set_param(gcb, 'nameOutportFuel_Massflow', ['Fuel_Massflow_' get_param(gcb, 'blockName')])
      | set_param(gcb, 'setOutportEngine_Speed', 'off')
      | set_param(gcb, 'nameOutportEngine_Speed', ['Omega_' get_param(gcb, 'blockName')])
      | set_param(gcb, 'setOutportCylinder_Pressure', 'off')
      | set_param(gcb, 'nameOutportCylinder_Pressure', ['Pressure_in_cylinder_' get_param(gcb, 'blockName')])
      settings: NameChangeFcn=|
      | %if variable name is default change this name on name change of block
      | 
      | 
      | if strcmp(get_param(gcb, 'nameOutportFuel_Massflow'), [ 'Fuel_Massflow_' get_param(gcb, 'blockName') ])
      | set_param(gcb, 'nameOutportFuel_Massflow', ['Fuel_Massflow_' get_param(gcb, 'Name')])
      | end
      | 
      | 
      | 
      | 
      | if strcmp(get_param(gcb, 'nameOutportEngine_Speed'), [ 'Omega_' get_param(gcb, 'blockName') ])
      | set_param(gcb, 'nameOutportEngine_Speed', ['Omega_' get_param(gcb, 'Name')])
      | end
      | 
      | 
      | set_param(gcb, 'blockName', get_param(gcb, 'Name'))
      mask CallbackString:
      | en = get_param(gcb,'MaskEnables');
      | 
      | switch get_param(gcb,'setOutportFuel_Massflow')
      | 
      |     case 'on'
      |         en{2} = 'on';
      |     case 'off'
      |         en{2} = 'off';
      | end
      | 
      | set_param(gcb,'MaskEnables',en)|%% Check for empty strings
      | if isempty(strtrim(get_param(gcb, 'nameOutportFuel_Massflow')))
      |     set_param(gcb, 'nameOutportFuel_Massflow', ['Fuel_Massflow_' get_param(gcb, 'Name')])
      |     error('Empty string for readout variable not allowed')
      | end
      | 
      | 
      | %% Check for repeated outport names
      | checkOutportName('nameOutportFuel_Massflow', 'Fuel_Massflow')|en = get_param(gcb,'MaskEnables');
      | 
      | switch get_param(gcb,'setOutportEngine_Speed')
      | 
      |     case 'on'
      |         en{4} = 'on';
      |     case 'off'
      |         en{4} = 'off';
      | end
      | 
      | set_param(gcb,'MaskEnables',en)|%% Check for empty strings
      | if isempty(strtrim(get_param(gcb, 'nameOutportEngine_Speed')))
      |     set_param(gcb, 'nameOutportEngine_Speed', ['Engine_Speed_' get_param(gcb, 'Name')])
      |     error('Empty string for readout variable not allowed')
      | end
      | 
      | 
      | %% Check for repeated outport names
      | checkOutportName('nameOutportEngine_Speed', 'Engine_Speed')|en = get_param(gcb,'MaskEnables');
      | 
      | switch get_param(gcb,'setOutportCylinder_Pressure')
      | 
      |     case 'on'
      |         en{6} = 'on';
      |     case 'off'
      |         en{6} = 'off';
      | end
      | 
      | set_param(gcb,'MaskEnables',en)|%% Check for empty strings
      | if isempty(strtrim(get_param(gcb, 'nameOutportFuel_Massflow')))
      |     set_param(gcb, 'nameOutportFuel_Massflow', ['Fuel_Massflow_' get_param(gcb, 'Name')])
      |     error('Empty string for readout variable not allowed')
      | end
      | 
      | 
      | %% Check for repeated outport names
      | checkOutportName('nameOutportFuel_Massflow', 'Fuel_Massflow')|
      mask Display:
      | plot([-0.1], [-0.1])
      | plot([1.1], [1.1])
      | plot([0.18,0.18],[0,1])
      | plot([0.21,0.21],[0,1])
      | plot([0.82,0.82],[0,1])
      | plot([0.79,0.79],[0,1])
      | plot([0.22,0.22,0.3, 0.7, 0.78, 0.78, 0.22],[0.8, 0.4, 0.35, 0.35, 0.4,0.8,0.8])
      | plot([0.21,0.79],[0.7,0.7])
      | plot([0.21,0.79],[0.66,0.66])
      | plot([0.21,0.79],[0.7,0.7])
      | plot([0.47,0.6],[0.35,0])
      | plot([0.53,0.66],[0.35,0])
      | 
      | color('green');
      | plot(xSpeed1, ySpeed1)
      | plot(xSpeed2, ySpeed2)
      | plot(xSpeed3, ySpeed3)
      | 
      | color('magenta');
      | plot(xFlow1, yFlow1)
      | plot(xFlow2, yFlow2)
      | plot(xFlow3, yFlow3)
      | plot(xFlow4, yFlow4)
      | 
      | color('blue');
      | plot(xPress1, yPress1)
      | plot(xPress2, yPress2)
      | plot(xPress3, yPress3)
      | plot(xPress4, yPress4)
  Engine9 : Subsystem  mask(engine_subsys){setOutportFuel_Massflow=off, nameOutportFuel_Massflow=Fuel_Massflow_Engine9, setOutportEngine_Speed=off, nameOutportEngine_Speed=Omega_Engine9, setOutportCylinder_Pressure=off, nameOutportCylinder_Pressure=Pressure_in_cylinder_Engine9, blockName=Engine9}
      mask prompts: setOutportFuel_Massflow "readout fuel mass flow [kg/s]"; nameOutportFuel_Massflow "variable name to readout fuel mass flow"; setOutportEngine_Speed "readout engine speed [rad/s]"; nameOutportEngine_Speed "variable name to readout engine speed"; setOutportCylinder_Pressure "readout cylinder pressure [Pa]"; nameOutportCylinder_Pressure "variable name to readout cylinder pressure"; blockName "name of readout block (internal use only)"
      mask init: same as Supported_and_unsupported_combinations/Engine
      settings: CopyFcn=|
      | set_param(gcb, 'blockName', get_param(gcb, 'Name'))
      | set_param(gcb, 'setOutportFuel_Massflow', 'off')
      | set_param(gcb, 'nameOutportFuel_Massflow', ['Fuel_Massflow_' get_param(gcb, 'blockName')])
      | set_param(gcb, 'setOutportEngine_Speed', 'off')
      | set_param(gcb, 'nameOutportEngine_Speed', ['Omega_' get_param(gcb, 'blockName')])
      | set_param(gcb, 'setOutportCylinder_Pressure', 'off')
      | set_param(gcb, 'nameOutportCylinder_Pressure', ['Pressure_in_cylinder_' get_param(gcb, 'blockName')])
      settings: NameChangeFcn=|
      | %if variable name is default change this name on name change of block
      | 
      | 
      | if strcmp(get_param(gcb, 'nameOutportFuel_Massflow'), [ 'Fuel_Massflow_' get_param(gcb, 'blockName') ])
      | set_param(gcb, 'nameOutportFuel_Massflow', ['Fuel_Massflow_' get_param(gcb, 'Name')])
      | end
      | 
      | 
      | 
      | 
      | if strcmp(get_param(gcb, 'nameOutportEngine_Speed'), [ 'Omega_' get_param(gcb, 'blockName') ])
      | set_param(gcb, 'nameOutportEngine_Speed', ['Omega_' get_param(gcb, 'Name')])
      | end
      | 
      | 
      | set_param(gcb, 'blockName', get_param(gcb, 'Name'))
      mask CallbackString:
      | en = get_param(gcb,'MaskEnables');
      | 
      | switch get_param(gcb,'setOutportFuel_Massflow')
      | 
      |     case 'on'
      |         en{2} = 'on';
      |     case 'off'
      |         en{2} = 'off';
      | end
      | 
      | set_param(gcb,'MaskEnables',en)|%% Check for empty strings
      | if isempty(strtrim(get_param(gcb, 'nameOutportFuel_Massflow')))
      |     set_param(gcb, 'nameOutportFuel_Massflow', ['Fuel_Massflow_' get_param(gcb, 'Name')])
      |     error('Empty string for readout variable not allowed')
      | end
      | 
      | 
      | %% Check for repeated outport names
      | checkOutportName('nameOutportFuel_Massflow', 'Fuel_Massflow')|en = get_param(gcb,'MaskEnables');
      | 
      | switch get_param(gcb,'setOutportEngine_Speed')
      | 
      |     case 'on'
      |         en{4} = 'on';
      |     case 'off'
      |         en{4} = 'off';
      | end
      | 
      | set_param(gcb,'MaskEnables',en)|%% Check for empty strings
      | if isempty(strtrim(get_param(gcb, 'nameOutportEngine_Speed')))
      |     set_param(gcb, 'nameOutportEngine_Speed', ['Engine_Speed_' get_param(gcb, 'Name')])
      |     error('Empty string for readout variable not allowed')
      | end
      | 
      | 
      | %% Check for repeated outport names
      | checkOutportName('nameOutportEngine_Speed', 'Engine_Speed')|en = get_param(gcb,'MaskEnables');
      | 
      | switch get_param(gcb,'setOutportCylinder_Pressure')
      | 
      |     case 'on'
      |         en{6} = 'on';
      |     case 'off'
      |         en{6} = 'off';
      | end
      | 
      | set_param(gcb,'MaskEnables',en)|%% Check for empty strings
      | if isempty(strtrim(get_param(gcb, 'nameOutportFuel_Massflow')))
      |     set_param(gcb, 'nameOutportFuel_Massflow', ['Fuel_Massflow_' get_param(gcb, 'Name')])
      |     error('Empty string for readout variable not allowed')
      | end
      | 
      | 
      | %% Check for repeated outport names
      | checkOutportName('nameOutportFuel_Massflow', 'Fuel_Massflow')|
      mask Display:
      | plot([-0.1], [-0.1])
      | plot([1.1], [1.1])
      | plot([0.18,0.18],[0,1])
      | plot([0.21,0.21],[0,1])
      | plot([0.82,0.82],[0,1])
      | plot([0.79,0.79],[0,1])
      | plot([0.22,0.22,0.3, 0.7, 0.78, 0.78, 0.22],[0.8, 0.4, 0.35, 0.35, 0.4,0.8,0.8])
      | plot([0.21,0.79],[0.7,0.7])
      | plot([0.21,0.79],[0.66,0.66])
      | plot([0.21,0.79],[0.7,0.7])
      | plot([0.47,0.6],[0.35,0])
      | plot([0.53,0.66],[0.35,0])
      | 
      | color('green');
      | plot(xSpeed1, ySpeed1)
      | plot(xSpeed2, ySpeed2)
      | plot(xSpeed3, ySpeed3)
      | 
      | color('magenta');
      | plot(xFlow1, yFlow1)
      | plot(xFlow2, yFlow2)
      | plot(xFlow3, yFlow3)
      | plot(xFlow4, yFlow4)
      | 
      | color('blue');
      | plot(xPress1, yPress1)
      | plot(xPress2, yPress2)
      | plot(xPress3, yPress3)
      | plot(xPress4, yPress4)
  FlowRestriction : Subsystem  mask{FlowRestriction=off}
      mask Display:
      | plot([0], [0])
      | plot([1], [1])
      | plot([0.1 0.9 0.1 0.9 0.1], [0.1 0.1 0.9 0.9 0.1])
  FlowRestriction1 : Subsystem  mask{FlowRestriction=off}
      mask Display:
      | plot([0], [0])
      | plot([1], [1])
      | plot([0.1 0.9 0.1 0.9 0.1], [0.1 0.1 0.9 0.9 0.1])
  FlowRestriction2 : Subsystem  mask{FlowRestriction=off}
      mask Display:
      | plot([0], [0])
      | plot([1], [1])
      | plot([0.1 0.9 0.1 0.9 0.1], [0.1 0.1 0.9 0.9 0.1])
  FlowRestriction3 : Subsystem  mask{FlowRestriction=off}
      mask Display:
      | plot([0], [0])
      | plot([1], [1])
      | plot([0.1 0.9 0.1 0.9 0.1], [0.1 0.1 0.9 0.9 0.1])
  FlowRestriction4 : Subsystem  mask{FlowRestriction=off}
      mask Display:
      | plot([0], [0])
      | plot([1], [1])
      | plot([0.1 0.9 0.1 0.9 0.1], [0.1 0.1 0.9 0.9 0.1])
  FlowRestriction5 : Subsystem  mask{FlowRestriction=off}
      mask Display:
      | plot([0], [0])
      | plot([1], [1])
      | plot([0.1 0.9 0.1 0.9 0.1], [0.1 0.1 0.9 0.9 0.1])
  FlowRestriction6 : Subsystem  mask{FlowRestriction=off}
      mask Display:
      | plot([0], [0])
      | plot([1], [1])
      | plot([0.1 0.9 0.1 0.9 0.1], [0.1 0.1 0.9 0.9 0.1])
  FlowRestriction7 : Subsystem  mask{FlowRestriction=off}
      mask Display:
      | plot([0], [0])
      | plot([1], [1])
      | plot([0.1 0.9 0.1 0.9 0.1], [0.1 0.1 0.9 0.9 0.1])
  FlowSplitter : Subsystem  mask{FlowSplitter=0}
      mask Display:
      | plot([0 1 1 0 0], [0 0 1 1 0])
      | plot([0.2 0.5], [0.5 0.5])
      | plot([0.5 0.5], [0.2 0.8])
      | plot([0.5 0.8], [0.8 0.8])
      | plot([0.5 0.8], [0.2 0.2])
  FlowSplitter1 : Subsystem  mask{FlowSplitter=0}
      mask Display:
      | plot([0 1 1 0 0], [0 0 1 1 0])
      | plot([0.2 0.5], [0.5 0.5])
      | plot([0.5 0.5], [0.2 0.8])
      | plot([0.5 0.8], [0.8 0.8])
      | plot([0.5 0.8], [0.2 0.2])
  FlowSplitter2 : Subsystem  mask{FlowSplitter=0}
      mask Display:
      | plot([0 1 1 0 0], [0 0 1 1 0])
      | plot([0.2 0.5], [0.5 0.5])
      | plot([0.5 0.5], [0.2 0.8])
      | plot([0.5 0.8], [0.8 0.8])
      | plot([0.5 0.8], [0.2 0.2])
  FlowSplitter3 : Subsystem  mask{FlowSplitter=0}
      mask Display:
      | plot([0 1 1 0 0], [0 0 1 1 0])
      | plot([0.2 0.5], [0.5 0.5])
      | plot([0.5 0.5], [0.2 0.8])
      | plot([0.5 0.8], [0.8 0.8])
      | plot([0.5 0.8], [0.2 0.2])
  HeatExchanger : Subsystem  mask{HeatExchanger=0}
      mask Display: plot([0.1 0.1 0.2 0.3 0.4 0.5 0.6 0.7 0.8 0.9 0.9], [1 0 0.6 0 0.6 0 0.6 0 0.6 0 1])
  HeatExchanger1 : Subsystem  mask{HeatExchanger=0}
      mask Display: plot([0.1 0.1 0.2 0.3 0.4 0.5 0.6 0.7 0.8 0.9 0.9], [1 0 0.6 0 0.6 0 0.6 0 0.6 0 1])
  HeatExchanger2 : Subsystem  mask{HeatExchanger=0}
      mask Display: plot([0.1 0.1 0.2 0.3 0.4 0.5 0.6 0.7 0.8 0.9 0.9], [1 0 0.6 0 0.6 0 0.6 0 0.6 0 1])
  HeatExchanger3 : Subsystem  mask{HeatExchanger=0}
      mask Display: plot([0.1 0.1 0.2 0.3 0.4 0.5 0.6 0.7 0.8 0.9 0.9], [1 0 0.6 0 0.6 0 0.6 0 0.6 0 1])
  Mix : Subsystem  mask{Mix=0}
      mask Display:
      | plot([0 1 1 0 0], [0 0 1 1 0])
      | plot([0.5 0.5], [1 0.8])
      | plot([0.4 0.6 0.6 0.4 0.4], [0.7 0.9 0.7 0.9 0.7])
  Mix1 : Subsystem  mask{Mix=0}
      mask Display:
      | plot([0 1 1 0 0], [0 0 1 1 0])
      | plot([0.5 0.5], [1 0.8])
      | plot([0.4 0.6 0.6 0.4 0.4], [0.7 0.9 0.7 0.9 0.7])
  Mix2 : Subsystem  mask{Mix=0}
      mask Display:
      | plot([0 1 1 0 0], [0 0 1 1 0])
      | plot([0.5 0.5], [1 0.8])
      | plot([0.4 0.6 0.6 0.4 0.4], [0.7 0.9 0.7 0.9 0.7])
  Mix3 : Subsystem  mask{Mix=0}
      mask Display:
      | plot([0 1 1 0 0], [0 0 1 1 0])
      | plot([0.5 0.5], [1 0.8])
      | plot([0.4 0.6 0.6 0.4 0.4], [0.7 0.9 0.7 0.9 0.7])
  UnitConversion1 : S-Function  Tag=conversionblock  FunctionName=orsb_signal_conversion  Parameters=convCategory, convType, convScale, convOffset, isOutput  EnableBusSupport=off  mask{convCategory=injection, convType=not defined, convScale=1, convOffset=0, isOutput=off}
      mask prompts: convCategory "Signal Category"; convType "Units"; convScale "Scale"; convOffset "Offset"; isOutput "use for ouput conversion"
      mask init:
      | try 
      | 
      |     %succeeds if conversion table defined in base workspace
      |     orsb_ConversionTable = evalin('base', 'orsb_ConversionTable');
      | 
      | catch exception
      |     
      |     curSys = strtok(gcs, '/');
      | 
      |     orsb_ConversionTable = get_param(curSys, 'Metadata');
      |     
      | end
      | 
      | if ~isempty(orsb_ConversionTable)
      |     
      |     numEntries = numel(orsb_ConversionTable);
      | 
      |     for i= 1 : numEntries
      |         listCategory{i} = orsb_ConversionTable(i).category;
      |         listConversion{i} = orsb_ConversionTable(i).name;
      |         listScale(i) = orsb_ConversionTable(i).scale;
      |         listOffset(i) = orsb_ConversionTable(i).offset;
      |     end
      | 
      |     %find matching entry in conversion table
      |     idxUnitsMatch = find(strcmp(convCategory, listCategory) & strcmp(convType, listConversion));
      |     switch numel(idxUnitsMatch)
      |         case 0 %no match found
      |             convType = 'not defined';
      |             convScale  = 1;
      |             convOffset = 0;
      |         case 1
      |             if ~isOutput
      |                 convScale = listScale(idxUnitsMatch);
      |                 convOffset = listOffset(idxUnitsMatch);
      |             else
      |                 convScale = 1 / listScale(idxUnitsMatch);
      |                 convOffset = -listOffset(idxUnitsMatch) / listScale(idxUnitsMatch);
      |             end
      |         otherwise % more than one match found
      |             error('Units entered multiple times.')
      |     end
      | 
      |     %writing parameters with set_param seems required to permanently overwrite values
      |     set_param(gcb, 'convScale', num2str(convScale)) 
      |     set_param(gcb, 'convOffset', num2str(convOffset))
      |     set_param(gcb, 'convType', convType)
      | 
      | end
      settings: OpenFcn=setUnitConverstionBlockInterface([], gcb)
      mask Display:
      | plot(0, 0)
      | plot(1, 1)
      | plot([0, 1], [0.5, 0.5])
      | plot([0.4 0.6], [0.1 0.9])
  UnitConversion10 : S-Function  Tag=conversionblock  FunctionName=orsb_signal_conversion  Parameters=convCategory, convType, convScale, convOffset, isOutput  EnableBusSupport=off  mask{convCategory=speed, convType=not defined, convScale=1, convOffset=0, isOutput=off}
      mask prompts: convCategory "Signal Category"; convType "Units"; convScale "Scale"; convOffset "Offset"; isOutput "use for ouput conversion"
      mask init: same as Supported_and_unsupported_combinations/UnitConversion1
      settings: OpenFcn=setUnitConverstionBlockInterface([], gcb)
      mask Display:
      | plot(0, 0)
      | plot(1, 1)
      | plot([0, 1], [0.5, 0.5])
      | plot([0.4 0.6], [0.1 0.9])
  UnitConversion11 : S-Function  Tag=conversionblock  FunctionName=orsb_signal_conversion  Parameters=convCategory, convType, convScale, convOffset, isOutput  EnableBusSupport=off  mask{convCategory=timing, convType=not defined, convScale=1, convOffset=0, isOutput=off}
      mask prompts: convCategory "Signal Category"; convType "Units"; convScale "Scale"; convOffset "Offset"; isOutput "use for ouput conversion"
      mask init: same as Supported_and_unsupported_combinations/UnitConversion1
      settings: OpenFcn=setUnitConverstionBlockInterface([], gcb)
      mask Display:
      | plot(0, 0)
      | plot(1, 1)
      | plot([0, 1], [0.5, 0.5])
      | plot([0.4 0.6], [0.1 0.9])
  UnitConversion12 : S-Function  Tag=conversionblock  FunctionName=orsb_signal_conversion  Parameters=convCategory, convType, convScale, convOffset, isOutput  EnableBusSupport=off  mask{convCategory=pressure, convType=not defined, convScale=1, convOffset=0, isOutput=off}
      mask prompts: convCategory "Signal Category"; convType "Units"; convScale "Scale"; convOffset "Offset"; isOutput "use for ouput conversion"
      mask init: same as Supported_and_unsupported_combinations/UnitConversion1
      settings: OpenFcn=setUnitConverstionBlockInterface([], gcb)
      mask Display:
      | plot(0, 0)
      | plot(1, 1)
      | plot([0, 1], [0.5, 0.5])
      | plot([0.4 0.6], [0.1 0.9])
  UnitConversion13 : S-Function  Tag=conversionblock  FunctionName=orsb_signal_conversion  Parameters=convCategory, convType, convScale, convOffset, isOutput  EnableBusSupport=off  mask{convCategory=timing, convType=not defined, convScale=1, convOffset=0, isOutput=off}
      mask prompts: convCategory "Signal Category"; convType "Units"; convScale "Scale"; convOffset "Offset"; isOutput "use for ouput conversion"
      mask init: same as Supported_and_unsupported_combinations/UnitConversion1
      settings: OpenFcn=setUnitConverstionBlockInterface([], gcb)
      mask Display:
      | plot(0, 0)
      | plot(1, 1)
      | plot([0, 1], [0.5, 0.5])
      | plot([0.4 0.6], [0.1 0.9])
  UnitConversion14 : S-Function  Tag=conversionblock  FunctionName=orsb_signal_conversion  Parameters=convCategory, convType, convScale, convOffset, isOutput  EnableBusSupport=off  mask{convCategory=injection, convType=not defined, convScale=1, convOffset=0, isOutput=off}
      mask prompts: convCategory "Signal Category"; convType "Units"; convScale "Scale"; convOffset "Offset"; isOutput "use for ouput conversion"
      mask init: same as Supported_and_unsupported_combinations/UnitConversion1
      settings: OpenFcn=setUnitConverstionBlockInterface([], gcb)
      mask Display:
      | plot(0, 0)
      | plot(1, 1)
      | plot([0, 1], [0.5, 0.5])
      | plot([0.4 0.6], [0.1 0.9])
  UnitConversion15 : S-Function  Tag=conversionblock  FunctionName=orsb_signal_conversion  Parameters=convCategory, convType, convScale, convOffset, isOutput  EnableBusSupport=off  mask{convCategory=speed, convType=not defined, convScale=1, convOffset=0, isOutput=off}
      mask prompts: convCategory "Signal Category"; convType "Units"; convScale "Scale"; convOffset "Offset"; isOutput "use for ouput conversion"
      mask init: same as Supported_and_unsupported_combinations/UnitConversion1
      settings: OpenFcn=setUnitConverstionBlockInterface([], gcb)
      mask Display:
      | plot(0, 0)
      | plot(1, 1)
      | plot([0, 1], [0.5, 0.5])
      | plot([0.4 0.6], [0.1 0.9])
  UnitConversion16 : S-Function  Tag=conversionblock  FunctionName=orsb_signal_conversion  Parameters=convCategory, convType, convScale, convOffset, isOutput  EnableBusSupport=off  mask{convCategory=pressure, convType=not defined, convScale=1, convOffset=0, isOutput=off}
      mask prompts: convCategory "Signal Category"; convType "Units"; convScale "Scale"; convOffset "Offset"; isOutput "use for ouput conversion"
      mask init: same as Supported_and_unsupported_combinations/UnitConversion1
      settings: OpenFcn=setUnitConverstionBlockInterface([], gcb)
      mask Display:
      | plot(0, 0)
      | plot(1, 1)
      | plot([0, 1], [0.5, 0.5])
      | plot([0.4 0.6], [0.1 0.9])
  UnitConversion17 : S-Function  Tag=conversionblock  FunctionName=orsb_signal_conversion  Parameters=convCategory, convType, convScale, convOffset, isOutput  EnableBusSupport=off  mask{convCategory=timing, convType=not defined, convScale=1, convOffset=0, isOutput=off}
      mask prompts: convCategory "Signal Category"; convType "Units"; convScale "Scale"; convOffset "Offset"; isOutput "use for ouput conversion"
      mask init: same as Supported_and_unsupported_combinations/UnitConversion1
      settings: OpenFcn=setUnitConverstionBlockInterface([], gcb)
      mask Display:
      | plot(0, 0)
      | plot(1, 1)
      | plot([0, 1], [0.5, 0.5])
      | plot([0.4 0.6], [0.1 0.9])
  UnitConversion18 : S-Function  Tag=conversionblock  FunctionName=orsb_signal_conversion  Parameters=convCategory, convType, convScale, convOffset, isOutput  EnableBusSupport=off  mask{convCategory=injection, convType=not defined, convScale=1, convOffset=0, isOutput=off}
      mask prompts: convCategory "Signal Category"; convType "Units"; convScale "Scale"; convOffset "Offset"; isOutput "use for ouput conversion"
      mask init: same as Supported_and_unsupported_combinations/UnitConversion1
      settings: OpenFcn=setUnitConverstionBlockInterface([], gcb)
      mask Display:
      | plot(0, 0)
      | plot(1, 1)
      | plot([0, 1], [0.5, 0.5])
      | plot([0.4 0.6], [0.1 0.9])
  UnitConversion19 : S-Function  Tag=conversionblock  FunctionName=orsb_signal_conversion  Parameters=convCategory, convType, convScale, convOffset, isOutput  EnableBusSupport=off  mask{convCategory=speed, convType=not defined, convScale=1, convOffset=0, isOutput=off}
      mask prompts: convCategory "Signal Category"; convType "Units"; convScale "Scale"; convOffset "Offset"; isOutput "use for ouput conversion"
      mask init: same as Supported_and_unsupported_combinations/UnitConversion1
      settings: OpenFcn=setUnitConverstionBlockInterface([], gcb)
      mask Display:
      | plot(0, 0)
      | plot(1, 1)
      | plot([0, 1], [0.5, 0.5])
      | plot([0.4 0.6], [0.1 0.9])
  UnitConversion2 : S-Function  Tag=conversionblock  FunctionName=orsb_signal_conversion  Parameters=convCategory, convType, convScale, convOffset, isOutput  EnableBusSupport=off  mask{convCategory=timing, convType=not defined, convScale=1, convOffset=0, isOutput=off}
      mask prompts: convCategory "Signal Category"; convType "Units"; convScale "Scale"; convOffset "Offset"; isOutput "use for ouput conversion"
      mask init: same as Supported_and_unsupported_combinations/UnitConversion1
      settings: OpenFcn=setUnitConverstionBlockInterface([], gcb)
      mask Display:
      | plot(0, 0)
      | plot(1, 1)
      | plot([0, 1], [0.5, 0.5])
      | plot([0.4 0.6], [0.1 0.9])
  UnitConversion20 : S-Function  Tag=conversionblock  FunctionName=orsb_signal_conversion  Parameters=convCategory, convType, convScale, convOffset, isOutput  EnableBusSupport=off  mask{convCategory=pressure, convType=not defined, convScale=1, convOffset=0, isOutput=off}
      mask prompts: convCategory "Signal Category"; convType "Units"; convScale "Scale"; convOffset "Offset"; isOutput "use for ouput conversion"
      mask init: same as Supported_and_unsupported_combinations/UnitConversion1
      settings: OpenFcn=setUnitConverstionBlockInterface([], gcb)
      mask Display:
      | plot(0, 0)
      | plot(1, 1)
      | plot([0, 1], [0.5, 0.5])
      | plot([0.4 0.6], [0.1 0.9])
  UnitConversion21 : S-Function  Tag=conversionblock  FunctionName=orsb_signal_conversion  Parameters=convCategory, convType, convScale, convOffset, isOutput  EnableBusSupport=off  mask{convCategory=timing, convType=not defined, convScale=1, convOffset=0, isOutput=off}
      mask prompts: convCategory "Signal Category"; convType "Units"; convScale "Scale"; convOffset "Offset"; isOutput "use for ouput conversion"
      mask init: same as Supported_and_unsupported_combinations/UnitConversion1
      settings: OpenFcn=setUnitConverstionBlockInterface([], gcb)
      mask Display:
      | plot(0, 0)
      | plot(1, 1)
      | plot([0, 1], [0.5, 0.5])
      | plot([0.4 0.6], [0.1 0.9])
  UnitConversion22 : S-Function  Tag=conversionblock  FunctionName=orsb_signal_conversion  Parameters=convCategory, convType, convScale, convOffset, isOutput  EnableBusSupport=off  mask{convCategory=injection, convType=not defined, convScale=1, convOffset=0, isOutput=off}
      mask prompts: convCategory "Signal Category"; convType "Units"; convScale "Scale"; convOffset "Offset"; isOutput "use for ouput conversion"
      mask init: same as Supported_and_unsupported_combinations/UnitConversion1
      settings: OpenFcn=setUnitConverstionBlockInterface([], gcb)
      mask Display:
      | plot(0, 0)
      | plot(1, 1)
      | plot([0, 1], [0.5, 0.5])
      | plot([0.4 0.6], [0.1 0.9])
  UnitConversion23 : S-Function  Tag=conversionblock  FunctionName=orsb_signal_conversion  Parameters=convCategory, convType, convScale, convOffset, isOutput  EnableBusSupport=off  mask{convCategory=speed, convType=not defined, convScale=1, convOffset=0, isOutput=off}
      mask prompts: convCategory "Signal Category"; convType "Units"; convScale "Scale"; convOffset "Offset"; isOutput "use for ouput conversion"
      mask init: same as Supported_and_unsupported_combinations/UnitConversion1
      settings: OpenFcn=setUnitConverstionBlockInterface([], gcb)
      mask Display:
      | plot(0, 0)
      | plot(1, 1)
      | plot([0, 1], [0.5, 0.5])
      | plot([0.4 0.6], [0.1 0.9])
  UnitConversion24 : S-Function  Tag=conversionblock  FunctionName=orsb_signal_conversion  Parameters=convCategory, convType, convScale, convOffset, isOutput  EnableBusSupport=off  mask{convCategory=pressure, convType=not defined, convScale=1, convOffset=0, isOutput=off}
      mask prompts: convCategory "Signal Category"; convType "Units"; convScale "Scale"; convOffset "Offset"; isOutput "use for ouput conversion"
      mask init: same as Supported_and_unsupported_combinations/UnitConversion1
      settings: OpenFcn=setUnitConverstionBlockInterface([], gcb)
      mask Display:
      | plot(0, 0)
      | plot(1, 1)
      | plot([0, 1], [0.5, 0.5])
      | plot([0.4 0.6], [0.1 0.9])
  UnitConversion25 : S-Function  Tag=conversionblock  FunctionName=orsb_signal_conversion  Parameters=convCategory, convType, convScale, convOffset, isOutput  EnableBusSupport=off  mask{convCategory=timing, convType=not defined, convScale=1, convOffset=0, isOutput=off}
      mask prompts: convCategory "Signal Category"; convType "Units"; convScale "Scale"; convOffset "Offset"; isOutput "use for ouput conversion"
      mask init: same as Supported_and_unsupported_combinations/UnitConversion1
      settings: OpenFcn=setUnitConverstionBlockInterface([], gcb)
      mask Display:
      | plot(0, 0)
      | plot(1, 1)
      | plot([0, 1], [0.5, 0.5])
      | plot([0.4 0.6], [0.1 0.9])
  UnitConversion26 : S-Function  Tag=conversionblock  FunctionName=orsb_signal_conversion  Parameters=convCategory, convType, convScale, convOffset, isOutput  EnableBusSupport=off  mask{convCategory=timing, convType=not defined, convScale=1, convOffset=0, isOutput=off}
      mask prompts: convCategory "Signal Category"; convType "Units"; convScale "Scale"; convOffset "Offset"; isOutput "use for ouput conversion"
      mask init: same as Supported_and_unsupported_combinations/UnitConversion1
      settings: OpenFcn=setUnitConverstionBlockInterface([], gcb)
      mask Display:
      | plot(0, 0)
      | plot(1, 1)
      | plot([0, 1], [0.5, 0.5])
      | plot([0.4 0.6], [0.1 0.9])
  UnitConversion27 : S-Function  Tag=conversionblock  FunctionName=orsb_signal_conversion  Parameters=convCategory, convType, convScale, convOffset, isOutput  EnableBusSupport=off  mask{convCategory=injection, convType=not defined, convScale=1, convOffset=0, isOutput=off}
      mask prompts: convCategory "Signal Category"; convType "Units"; convScale "Scale"; convOffset "Offset"; isOutput "use for ouput conversion"
      mask init: same as Supported_and_unsupported_combinations/UnitConversion1
      settings: OpenFcn=setUnitConverstionBlockInterface([], gcb)
      mask Display:
      | plot(0, 0)
      | plot(1, 1)
      | plot([0, 1], [0.5, 0.5])
      | plot([0.4 0.6], [0.1 0.9])
  UnitConversion28 : S-Function  Tag=conversionblock  FunctionName=orsb_signal_conversion  Parameters=convCategory, convType, convScale, convOffset, isOutput  EnableBusSupport=off  mask{convCategory=speed, convType=not defined, convScale=1, convOffset=0, isOutput=off}
      mask prompts: convCategory "Signal Category"; convType "Units"; convScale "Scale"; convOffset "Offset"; isOutput "use for ouput conversion"
      mask init: same as Supported_and_unsupported_combinations/UnitConversion1
      settings: OpenFcn=setUnitConverstionBlockInterface([], gcb)
      mask Display:
      | plot(0, 0)
      | plot(1, 1)
      | plot([0, 1], [0.5, 0.5])
      | plot([0.4 0.6], [0.1 0.9])
  UnitConversion29 : S-Function  Tag=conversionblock  FunctionName=orsb_signal_conversion  Parameters=convCategory, convType, convScale, convOffset, isOutput  EnableBusSupport=off  mask{convCategory=pressure, convType=not defined, convScale=1, convOffset=0, isOutput=off}
      mask prompts: convCategory "Signal Category"; convType "Units"; convScale "Scale"; convOffset "Offset"; isOutput "use for ouput conversion"
      mask init: same as Supported_and_unsupported_combinations/UnitConversion1
      settings: OpenFcn=setUnitConverstionBlockInterface([], gcb)
      mask Display:
      | plot(0, 0)
      | plot(1, 1)
      | plot([0, 1], [0.5, 0.5])
      | plot([0.4 0.6], [0.1 0.9])
  UnitConversion3 : S-Function  Tag=conversionblock  FunctionName=orsb_signal_conversion  Parameters=convCategory, convType, convScale, convOffset, isOutput  EnableBusSupport=off  mask{convCategory=injection, convType=not defined, convScale=1, convOffset=0, isOutput=off}
      mask prompts: convCategory "Signal Category"; convType "Units"; convScale "Scale"; convOffset "Offset"; isOutput "use for ouput conversion"
      mask init: same as Supported_and_unsupported_combinations/UnitConversion1
      settings: OpenFcn=setUnitConverstionBlockInterface([], gcb)
      mask Display:
      | plot(0, 0)
      | plot(1, 1)
      | plot([0, 1], [0.5, 0.5])
      | plot([0.4 0.6], [0.1 0.9])
  UnitConversion30 : S-Function  Tag=conversionblock  FunctionName=orsb_signal_conversion  Parameters=convCategory, convType, convScale, convOffset, isOutput  EnableBusSupport=off  mask{convCategory=timing, convType=not defined, convScale=1, convOffset=0, isOutput=off}
      mask prompts: convCategory "Signal Category"; convType "Units"; convScale "Scale"; convOffset "Offset"; isOutput "use for ouput conversion"
      mask init: same as Supported_and_unsupported_combinations/UnitConversion1
      settings: OpenFcn=setUnitConverstionBlockInterface([], gcb)
      mask Display:
      | plot(0, 0)
      | plot(1, 1)
      | plot([0, 1], [0.5, 0.5])
      | plot([0.4 0.6], [0.1 0.9])
  UnitConversion31 : S-Function  Tag=conversionblock  FunctionName=orsb_signal_conversion  Parameters=convCategory, convType, convScale, convOffset, isOutput  EnableBusSupport=off  mask{convCategory=injection, convType=not defined, convScale=1, convOffset=0, isOutput=off}
      mask prompts: convCategory "Signal Category"; convType "Units"; convScale "Scale"; convOffset "Offset"; isOutput "use for ouput conversion"
      mask init: same as Supported_and_unsupported_combinations/UnitConversion1
      settings: OpenFcn=setUnitConverstionBlockInterface([], gcb)
      mask Display:
      | plot(0, 0)
      | plot(1, 1)
      | plot([0, 1], [0.5, 0.5])
      | plot([0.4 0.6], [0.1 0.9])
  UnitConversion32 : S-Function  Tag=conversionblock  FunctionName=orsb_signal_conversion  Parameters=convCategory, convType, convScale, convOffset, isOutput  EnableBusSupport=off  mask{convCategory=speed, convType=not defined, convScale=1, convOffset=0, isOutput=off}
      mask prompts: convCategory "Signal Category"; convType "Units"; convScale "Scale"; convOffset "Offset"; isOutput "use for ouput conversion"
      mask init: same as Supported_and_unsupported_combinations/UnitConversion1
      settings: OpenFcn=setUnitConverstionBlockInterface([], gcb)
      mask Display:
      | plot(0, 0)
      | plot(1, 1)
      | plot([0, 1], [0.5, 0.5])
      | plot([0.4 0.6], [0.1 0.9])
  UnitConversion33 : S-Function  Tag=conversionblock  FunctionName=orsb_signal_conversion  Parameters=convCategory, convType, convScale, convOffset, isOutput  EnableBusSupport=off  mask{convCategory=pressure, convType=not defined, convScale=1, convOffset=0, isOutput=off}
      mask prompts: convCategory "Signal Category"; convType "Units"; convScale "Scale"; convOffset "Offset"; isOutput "use for ouput conversion"
      mask init: same as Supported_and_unsupported_combinations/UnitConversion1
      settings: OpenFcn=setUnitConverstionBlockInterface([], gcb)
      mask Display:
      | plot(0, 0)
      | plot(1, 1)
      | plot([0, 1], [0.5, 0.5])
      | plot([0.4 0.6], [0.1 0.9])
  UnitConversion34 : S-Function  Tag=conversionblock  FunctionName=orsb_signal_conversion  Parameters=convCategory, convType, convScale, convOffset, isOutput  EnableBusSupport=off  mask{convCategory=timing, convType=not defined, convScale=1, convOffset=0, isOutput=off}
      mask prompts: convCategory "Signal Category"; convType "Units"; convScale "Scale"; convOffset "Offset"; isOutput "use for ouput conversion"
      mask init: same as Supported_and_unsupported_combinations/UnitConversion1
      settings: OpenFcn=setUnitConverstionBlockInterface([], gcb)
      mask Display:
      | plot(0, 0)
      | plot(1, 1)
      | plot([0, 1], [0.5, 0.5])
      | plot([0.4 0.6], [0.1 0.9])
  UnitConversion35 : S-Function  Tag=conversionblock  FunctionName=orsb_signal_conversion  Parameters=convCategory, convType, convScale, convOffset, isOutput  EnableBusSupport=off  mask{convCategory=injection, convType=not defined, convScale=1, convOffset=0, isOutput=off}
      mask prompts: convCategory "Signal Category"; convType "Units"; convScale "Scale"; convOffset "Offset"; isOutput "use for ouput conversion"
      mask init: same as Supported_and_unsupported_combinations/UnitConversion1
      settings: OpenFcn=setUnitConverstionBlockInterface([], gcb)
      mask Display:
      | plot(0, 0)
      | plot(1, 1)
      | plot([0, 1], [0.5, 0.5])
      | plot([0.4 0.6], [0.1 0.9])
  UnitConversion36 : S-Function  Tag=conversionblock  FunctionName=orsb_signal_conversion  Parameters=convCategory, convType, convScale, convOffset, isOutput  EnableBusSupport=off  mask{convCategory=speed, convType=not defined, convScale=1, convOffset=0, isOutput=off}
      mask prompts: convCategory "Signal Category"; convType "Units"; convScale "Scale"; convOffset "Offset"; isOutput "use for ouput conversion"
      mask init: same as Supported_and_unsupported_combinations/UnitConversion1
      settings: OpenFcn=setUnitConverstionBlockInterface([], gcb)
      mask Display:
      | plot(0, 0)
      | plot(1, 1)
      | plot([0, 1], [0.5, 0.5])
      | plot([0.4 0.6], [0.1 0.9])
  UnitConversion37 : S-Function  Tag=conversionblock  FunctionName=orsb_signal_conversion  Parameters=convCategory, convType, convScale, convOffset, isOutput  EnableBusSupport=off  mask{convCategory=pressure, convType=not defined, convScale=1, convOffset=0, isOutput=off}
      mask prompts: convCategory "Signal Category"; convType "Units"; convScale "Scale"; convOffset "Offset"; isOutput "use for ouput conversion"
      mask init: same as Supported_and_unsupported_combinations/UnitConversion1
      settings: OpenFcn=setUnitConverstionBlockInterface([], gcb)
      mask Display:
      | plot(0, 0)
      | plot(1, 1)
      | plot([0, 1], [0.5, 0.5])
      | plot([0.4 0.6], [0.1 0.9])
  UnitConversion38 : S-Function  Tag=conversionblock  FunctionName=orsb_signal_conversion  Parameters=convCategory, convType, convScale, convOffset, isOutput  EnableBusSupport=off  mask{convCategory=injection, convType=not defined, convScale=1, convOffset=0, isOutput=off}
      mask prompts: convCategory "Signal Category"; convType "Units"; convScale "Scale"; convOffset "Offset"; isOutput "use for ouput conversion"
      mask init: same as Supported_and_unsupported_combinations/UnitConversion1
      settings: OpenFcn=setUnitConverstionBlockInterface([], gcb)
      mask Display:
      | plot(0, 0)
      | plot(1, 1)
      | plot([0, 1], [0.5, 0.5])
      | plot([0.4 0.6], [0.1 0.9])
  UnitConversion39 : S-Function  Tag=conversionblock  FunctionName=orsb_signal_conversion  Parameters=convCategory, convType, convScale, convOffset, isOutput  EnableBusSupport=off  mask{convCategory=speed, convType=not defined, convScale=1, convOffset=0, isOutput=off}
      mask prompts: convCategory "Signal Category"; convType "Units"; convScale "Scale"; convOffset "Offset"; isOutput "use for ouput conversion"
      mask init: same as Supported_and_unsupported_combinations/UnitConversion1
      settings: OpenFcn=setUnitConverstionBlockInterface([], gcb)
      mask Display:
      | plot(0, 0)
      | plot(1, 1)
      | plot([0, 1], [0.5, 0.5])
      | plot([0.4 0.6], [0.1 0.9])
  UnitConversion4 : S-Function  Tag=conversionblock  FunctionName=orsb_signal_conversion  Parameters=convCategory, convType, convScale, convOffset, isOutput  EnableBusSupport=off  mask{convCategory=speed, convType=not defined, convScale=1, convOffset=0, isOutput=off}
      mask prompts: convCategory "Signal Category"; convType "Units"; convScale "Scale"; convOffset "Offset"; isOutput "use for ouput conversion"
      mask init: same as Supported_and_unsupported_combinations/UnitConversion1
      settings: OpenFcn=setUnitConverstionBlockInterface([], gcb)
      mask Display:
      | plot(0, 0)
      | plot(1, 1)
      | plot([0, 1], [0.5, 0.5])
      | plot([0.4 0.6], [0.1 0.9])
  UnitConversion40 : S-Function  Tag=conversionblock  FunctionName=orsb_signal_conversion  Parameters=convCategory, convType, convScale, convOffset, isOutput  EnableBusSupport=off  mask{convCategory=pressure, convType=not defined, convScale=1, convOffset=0, isOutput=off}
      mask prompts: convCategory "Signal Category"; convType "Units"; convScale "Scale"; convOffset "Offset"; isOutput "use for ouput conversion"
      mask init: same as Supported_and_unsupported_combinations/UnitConversion1
      settings: OpenFcn=setUnitConverstionBlockInterface([], gcb)
      mask Display:
      | plot(0, 0)
      | plot(1, 1)
      | plot([0, 1], [0.5, 0.5])
      | plot([0.4 0.6], [0.1 0.9])
  UnitConversion5 : S-Function  Tag=conversionblock  FunctionName=orsb_signal_conversion  Parameters=convCategory, convType, convScale, convOffset, isOutput  EnableBusSupport=off  mask{convCategory=pressure, convType=not defined, convScale=1, convOffset=0, isOutput=off}
      mask prompts: convCategory "Signal Category"; convType "Units"; convScale "Scale"; convOffset "Offset"; isOutput "use for ouput conversion"
      mask init: same as Supported_and_unsupported_combinations/UnitConversion1
      settings: OpenFcn=setUnitConverstionBlockInterface([], gcb)
      mask Display:
      | plot(0, 0)
      | plot(1, 1)
      | plot([0, 1], [0.5, 0.5])
      | plot([0.4 0.6], [0.1 0.9])
  UnitConversion6 : S-Function  Tag=conversionblock  FunctionName=orsb_signal_conversion  Parameters=convCategory, convType, convScale, convOffset, isOutput  EnableBusSupport=off  mask{convCategory=timing, convType=not defined, convScale=1, convOffset=0, isOutput=off}
      mask prompts: convCategory "Signal Category"; convType "Units"; convScale "Scale"; convOffset "Offset"; isOutput "use for ouput conversion"
      mask init: same as Supported_and_unsupported_combinations/UnitConversion1
      settings: OpenFcn=setUnitConverstionBlockInterface([], gcb)
      mask Display:
      | plot(0, 0)
      | plot(1, 1)
      | plot([0, 1], [0.5, 0.5])
      | plot([0.4 0.6], [0.1 0.9])
  UnitConversion7 : S-Function  Tag=conversionblock  FunctionName=orsb_signal_conversion  Parameters=convCategory, convType, convScale, convOffset, isOutput  EnableBusSupport=off  mask{convCategory=injection, convType=not defined, convScale=1, convOffset=0, isOutput=off}
      mask prompts: convCategory "Signal Category"; convType "Units"; convScale "Scale"; convOffset "Offset"; isOutput "use for ouput conversion"
      mask init: same as Supported_and_unsupported_combinations/UnitConversion1
      settings: OpenFcn=setUnitConverstionBlockInterface([], gcb)
      mask Display:
      | plot(0, 0)
      | plot(1, 1)
      | plot([0, 1], [0.5, 0.5])
      | plot([0.4 0.6], [0.1 0.9])
  UnitConversion8 : S-Function  Tag=conversionblock  FunctionName=orsb_signal_conversion  Parameters=convCategory, convType, convScale, convOffset, isOutput  EnableBusSupport=off  mask{convCategory=speed, convType=not defined, convScale=1, convOffset=0, isOutput=off}
      mask prompts: convCategory "Signal Category"; convType "Units"; convScale "Scale"; convOffset "Offset"; isOutput "use for ouput conversion"
      mask init: same as Supported_and_unsupported_combinations/UnitConversion1
      settings: OpenFcn=setUnitConverstionBlockInterface([], gcb)
      mask Display:
      | plot(0, 0)
      | plot(1, 1)
      | plot([0, 1], [0.5, 0.5])
      | plot([0.4 0.6], [0.1 0.9])
  UnitConversion9 : S-Function  Tag=conversionblock  FunctionName=orsb_signal_conversion  Parameters=convCategory, convType, convScale, convOffset, isOutput  EnableBusSupport=off  mask{convCategory=pressure, convType=not defined, convScale=1, convOffset=0, isOutput=off}
      mask prompts: convCategory "Signal Category"; convType "Units"; convScale "Scale"; convOffset "Offset"; isOutput "use for ouput conversion"
      mask init: same as Supported_and_unsupported_combinations/UnitConversion1
      settings: OpenFcn=setUnitConverstionBlockInterface([], gcb)
      mask Display:
      | plot(0, 0)
      | plot(1, 1)
      | plot([0, 1], [0.5, 0.5])
      | plot([0.4 0.6], [0.1 0.9])
  wires:
  Neng/1 -> UnitConversion10/1
  IQ/1 -> UnitConversion1/1
  uSOI/1 -> UnitConversion2/1
  UnitConversion10/1 -> Engine/2(OmegaEng)
  UnitConversion1/1 -> Engine/3(IQ)
  UnitConversion2/1 -> Engine/4(uSOI)
  uPR/1 -> UnitConversion12/1
  UnitConversion12/1 -> Engine/5(uPR)
  BoundaryConditionsConstant/1(outflow) -> Engine/1(inflow)
  BoundaryConditionsConstant1/1(outflow) -> Mix/1(inflow1)
  BoundaryConditionsConstant2/1(outflow) -> HeatExchanger/1(inflow)
  Neng1/1 -> UnitConversion4/1
  IQ1/1 -> UnitConversion3/1
  uSOI1/1 -> UnitConversion6/1
  UnitConversion4/1 -> Engine1/2(OmegaEng)
  UnitConversion3/1 -> Engine1/3(IQ)
  UnitConversion6/1 -> Engine1/4(uSOI)
  uPR1/1 -> UnitConversion5/1
  UnitConversion5/1 -> Engine1/5(uPR)
  BoundaryConditionsConstant4/1(outflow) -> FlowRestriction1/1(inflow)
  BoundaryConditionsConstant5/1(outflow) -> FlowRestriction2/1(inflow)
  BoundaryConditionsConstant3/1(outflow) -> FlowRestriction/1(inflow)
  FlowRestriction/1(outflow) -> Engine1/1(inflow)
  FlowRestriction1/1(outflow) -> Mix1/1(inflow1)
  FlowRestriction2/1(outflow) -> HeatExchanger1/1(inflow)
  Neng2/1 -> UnitConversion8/1
  IQ2/1 -> UnitConversion7/1
  uSOI2/1 -> UnitConversion11/1
  UnitConversion8/1 -> Engine3/2(OmegaEng)
  UnitConversion7/1 -> Engine3/3(IQ)
  UnitConversion11/1 -> Engine3/4(uSOI)
  uPR2/1 -> UnitConversion9/1
  UnitConversion9/1 -> Engine3/5(uPR)
  Engine3/1(outflow) -> Mix2/1(inflow1)
  Neng3/1 -> UnitConversion15/1
  IQ3/1 -> UnitConversion14/1
  uSOI3/1 -> UnitConversion13/1
  UnitConversion15/1 -> Engine4/2(OmegaEng)
  UnitConversion14/1 -> Engine4/3(IQ)
  UnitConversion13/1 -> Engine4/4(uSOI)
  uPR3/1 -> UnitConversion16/1
  UnitConversion16/1 -> Engine4/5(uPR)
  Engine4/1(outflow) -> HeatExchanger2/1(inflow)
  Neng4/1 -> UnitConversion19/1
  IQ4/1 -> UnitConversion18/1
  uSOI4/1 -> UnitConversion17/1
  UnitConversion19/1 -> Engine5/2(OmegaEng)
  UnitConversion18/1 -> Engine5/3(IQ)
  UnitConversion17/1 -> Engine5/4(uSOI)
  uPR4/1 -> UnitConversion20/1
  UnitConversion20/1 -> Engine5/5(uPR)
  FlowSplitter/1(outflow1) -> Engine5/1(inflow)
  FlowSplitter1/1(outflow1) -> BoundaryConditionsConstant6/1(inflow)
  Neng5/1 -> UnitConversion23/1
  IQ5/1 -> UnitConversion22/1
  uSOI5/1 -> UnitConversion21/1
  UnitConversion23/1 -> Engine2/2(OmegaEng)
  UnitConversion22/1 -> Engine2/3(IQ)
  UnitConversion21/1 -> Engine2/4(uSOI)
  uPR5/1 -> UnitConversion24/1
  UnitConversion24/1 -> Engine2/5(uPR)
  Engine2/1(outflow) -> BoundaryConditionsConstant7/1(inflow)
  Neng6/1 -> UnitConversion39/1
  IQ6/1 -> UnitConversion38/1
  uSOI6/1 -> UnitConversion25/1
  UnitConversion39/1 -> Engine7/2(OmegaEng)
  UnitConversion38/1 -> Engine7/3(IQ)
  UnitConversion25/1 -> Engine7/4(uSOI)
  uPR6/1 -> UnitConversion40/1
  UnitConversion40/1 -> Engine7/5(uPR)
  Engine7/1(outflow) -> FlowRestriction4/1(inflow)
  Neng7/1 -> UnitConversion28/1
  IQ7/1 -> UnitConversion27/1
  uSOI7/1 -> UnitConversion26/1
  UnitConversion28/1 -> Engine8/2(OmegaEng)
  UnitConversion27/1 -> Engine8/3(IQ)
  UnitConversion26/1 -> Engine8/4(uSOI)
  uPR7/1 -> UnitConversion29/1
  UnitConversion29/1 -> Engine8/5(uPR)
  Engine8/1(outflow) -> FlowRestriction5/1(inflow)
  Neng8/1 -> UnitConversion32/1
  IQ8/1 -> UnitConversion31/1
  uSOI8/1 -> UnitConversion30/1
  UnitConversion32/1 -> Engine9/2(OmegaEng)
  UnitConversion31/1 -> Engine9/3(IQ)
  UnitConversion30/1 -> Engine9/4(uSOI)
  uPR8/1 -> UnitConversion33/1
  UnitConversion33/1 -> Engine9/5(uPR)
  FlowSplitter2/1(outflow1) -> FlowRestriction6/1(inflow)
  FlowSplitter3/1(outflow1) -> FlowRestriction7/1(inflow)
  Neng9/1 -> UnitConversion36/1
  IQ9/1 -> UnitConversion35/1
  uSOI9/1 -> UnitConversion34/1
  UnitConversion36/1 -> Engine6/2(OmegaEng)
  UnitConversion35/1 -> Engine6/3(IQ)
  UnitConversion34/1 -> Engine6/4(uSOI)
  uPR9/1 -> UnitConversion37/1
  UnitConversion37/1 -> Engine6/5(uPR)
  Engine6/1(outflow) -> FlowRestriction3/1(inflow)
  FlowRestriction3/1(outflow) -> BoundaryConditionsConstant9/1(inflow)
  FlowRestriction4/1(outflow) -> Mix3/1(inflow1)
  FlowRestriction5/1(outflow) -> HeatExchanger3/1(inflow)
  FlowRestriction6/1(outflow) -> Engine9/1(inflow)
  FlowRestriction7/1(outflow) -> BoundaryConditionsConstant8/1(inflow)
